simulink model "simu"  (R2019b)
settings: Solver=VariableStepAuto  StartTime=0.0  StopTime=1  RelTol=1e-3
(part 2 of 2)

== matlab function simu/Robot Torque  ==
  data: d1 input; te11 output; d2 input; d3 input; d4 input; L2 input; L3 input; L4 input; theta input; theta_dot input; theta_ddot input; mm input; II input; te22 output; te33 output; M output; G output; V output
function [te11,te22,te33,M,G,V] = fcn(d1,d2,d3,d4,L2,L3,L4,theta,theta_dot,theta_ddot,mm,II)
    theta1 = theta(1); theta2 = theta(2); theta3 = theta(3);
    theta1_dot = theta_dot(1); theta2_dot = theta_dot(2); theta3_dot = theta_dot(3);
    theta1_ddot = theta_ddot(1); theta2_ddot = theta_ddot(2); theta3_ddot = theta_ddot(3);
    m1 = mm(1); m2 =mm(2); m3 = mm(3); m4 = mm(4); m5 = mm(5);
    I1 = II(1); I2 = II(2); I3 = II(3); I4 = II(4); I5 = II(5);
    g = 9.8;
    te11 = 2*I1*theta1_ddot + 2*I2*theta1_ddot + 2*I3*theta1_ddot + 2*I4*theta1_ddot + 2*I5*theta1_ddot + (d2^2*m2*theta1_ddot)/2 + d2^2*m3*theta1_ddot + d2^2*m4*theta1_ddot + 2*d3^2*m3*theta1_ddot + d2^2*m5*theta1_ddot + d3^2*m4*theta1_ddot + d3^2*m5*theta1_ddot + 2*d4^2*m4*theta1_ddot + d4^2*m5*theta1_ddot + (5*L2^2*m3*theta1_ddot)/8 - (L2^2*m3*theta2_ddot)/4 + (L2^2*m4*theta1_ddot)/2 + (L2^2*m5*theta1_ddot)/2 + (5*L3^2*m4*theta1_ddot)/8 - (L3^2*m4*theta2_ddot)/4 + (L3^2*m5*theta1_ddot)/2 - (L3^2*m4*theta3_ddot)/4 + (5*L4^2*m5*theta1_ddot)/8 - (L4^2*m5*theta2_ddot)/4 - (L4^2*m5*theta3_ddot)/4 - (L2^2*m3*theta2_dot^2*sin(theta1 + theta2))/4 + (L3^2*m4*theta2_ddot*cos(theta1 + theta2 + theta3))/4 + (L3^2*m4*theta3_ddot*cos(theta1 + theta2 + theta3))/4 + (L4^2*m5*theta2_ddot*cos(theta1 + theta2 + theta3))/4 + (L4^2*m5*theta3_ddot*cos(theta1 + theta2 + theta3))/4 + (d2^2*m2*theta2_ddot*cos(theta1 - theta2))/2 - (d2^2*m2*theta2_dot^2*sin(theta1 + theta2))/2 - (d3^2*m3*theta1_dot^2*sin(theta1 + theta2))/2 + (L2^2*m3*theta1_ddot*cos(2*theta2))/2 + (L2^2*m4*theta1_ddot*cos(2*theta2))/2 + (L2^2*m5*theta1_ddot*cos(2*theta2))/2 + 2*d4^2*m4*theta1_ddot*cos(theta1 + theta2 + theta3) - (L2*g*m3*cos(theta1 + theta2))/2 - (L2*g*m4*cos(theta1 + theta2))/2 - (L2*g*m5*cos(theta1 + theta2))/2 + (d2^2*m2*theta1_ddot*cos(2*theta2))/2 - (d2*g*m2*sin(theta1 + theta2))/2 + (L2^2*m3*theta1_ddot*cos(2*theta2 + 2*theta3))/8 - (L2^2*m3*theta2_ddot*cos(2*theta2 + 2*theta3))/4 + (5*L3^2*m4*theta1_ddot*cos(2*theta2 + 2*theta3))/8 - (L3^2*m4*theta2_ddot*cos(2*theta2 + 2*theta3))/4 + (L3^2*m5*theta1_ddot*cos(2*theta2 + 2*theta3))/2 - (L3^2*m4*theta3_ddot*cos(2*theta2 + 2*theta3))/4 + (5*L4^2*m5*theta1_ddot*cos(2*theta2 + 2*theta3))/8 - (L4^2*m5*theta2_ddot*cos(2*theta2 + 2*theta3))/4 - (L4^2*m5*theta3_ddot*cos(2*theta2 + 2*theta3))/4 + (L2^2*m3*theta2_dot^2*sin(theta1 - theta2))/4 + (L3^2*m4*theta2_ddot*cos(theta2 - theta1 + theta3))/4 + (L3^2*m4*theta3_ddot*cos(theta2 - theta1 + theta3))/4 + (L4^2*m5*theta2_ddot*cos(theta2 - theta1 + theta3))/4 + (L4^2*m5*theta3_ddot*cos(theta2 - theta1 + theta3))/4 + (L2^2*m3*theta2_dot^2*sin(theta1 + theta2 + theta3))/4 + (d2^2*m2*theta2_dot^2*sin(theta1 - theta2))/2 - d2*g*m2*sin(theta1) - d2*g*m3*sin(theta1) - d2*g*m4*sin(theta1) - 2*d3*g*m3*sin(theta1) - d2*g*m5*sin(theta1) - d3*g*m4*sin(theta1) - d3*g*m5*sin(theta1) - 2*d4*g*m4*sin(theta1) - d4*g*m5*sin(theta1) + d3^2*m3*theta1_ddot*cos(theta1 + theta2 + 2*theta3) - (L2*g*m3*cos(theta1 - theta2))/2 - (L2*g*m4*cos(theta1 - theta2))/2 - (L2*g*m5*cos(theta1 - theta2))/2 - d4^2*m4*theta1_dot^2*sin(theta1 + theta2 + theta3) + (L2^2*m3*theta2_ddot*cos(theta1 + theta2))/4 + (L2^2*m3*theta3_ddot*cos(theta1 + theta2))/4 - (L2*g*m3*cos(theta1 + theta2 + theta3))/4 - (3*L3*g*m4*cos(theta1 + theta2 + theta3))/4 - (L3*g*m5*cos(theta1 + theta2 + theta3))/2 - (3*L4*g*m5*cos(theta1 + theta2 + theta3))/4 + (d2^2*m2*theta2_ddot*cos(theta1 + theta2))/2 + d3^2*m3*theta1_ddot*cos(theta1 + theta2) + (d2*g*m2*sin(theta1 - theta2))/2 + (L2^2*m3*theta2_dot^2*sin(2*theta2 + 2*theta3))/2 + (L3^2*m4*theta2_dot^2*sin(2*theta2 + 2*theta3))/2 + (L3^2*m4*theta3_dot^2*sin(2*theta2 + 2*theta3))/2 + (L4^2*m5*theta2_dot^2*sin(2*theta2 + 2*theta3))/2 + (L4^2*m5*theta3_dot^2*sin(2*theta2 + 2*theta3))/2 - (L2*L3*m4*theta2_ddot)/4 - (L2*L4*m5*theta2_ddot)/4 + L3*L4*m5*theta1_ddot - (L3*L4*m5*theta2_ddot)/4 - (L3*L4*m5*theta3_ddot)/4 + (L2^2*m3*theta2_dot^2*sin(theta2 - theta1 + theta3))/4 - (d3^2*m3*theta1_dot^2*sin(theta1 + theta2 + 2*theta3))/2 + (L2^2*m3*theta2_ddot*cos(theta1 - theta2))/4 + (L2^2*m3*theta3_ddot*cos(theta1 - theta2))/4 - (L2*g*m3*cos(theta2 - theta1 + theta3))/4 - (3*L3*g*m4*cos(theta2 - theta1 + theta3))/4 - (L3*g*m5*cos(theta2 - theta1 + theta3))/2 - (3*L4*g*m5*cos(theta2 - theta1 + theta3))/4 - d3^2*m3*theta1_dot*theta2_dot*sin(theta1 + theta2 + 2*theta3) - 2*d3^2*m3*theta1_dot*theta3_dot*sin(theta1 + theta2 + 2*theta3) + (L2*d2*m3*theta2_ddot*sin(theta1 - theta2))/4 + (L2*d2*m3*theta3_ddot*sin(theta1 - theta2))/4 - (L2*d2*m3*theta1_ddot*sin(2*theta2 + theta3))/2 + (L2*d3*m3*theta2_ddot*sin(theta1 - theta3))/4 + (L3*d2*m4*theta2_ddot*sin(theta1 - theta2))/4 - (L2*d3*m3*theta1_ddot*sin(theta2 + 2*theta3))/2 + (L2*d3*m3*theta3_ddot*sin(theta1 - theta3))/4 + (L3*d2*m4*theta3_ddot*sin(theta1 - theta2))/4 - (L3*d2*m4*theta1_ddot*sin(2*theta2 + theta3))/2 + (L3*d3*m4*theta2_ddot*sin(theta1 - theta3))/4 + (L4*d2*m5*theta2_ddot*sin(theta1 - theta2))/4 - (L3*d3*m4*theta1_ddot*sin(theta2 + 2*theta3))/2 + (L3*d3*m4*theta3_ddot*sin(theta1 - theta3))/4 + (L4*d2*m5*theta3_ddot*sin(theta1 - theta2))/4 - (L4*d2*m5*theta1_ddot*sin(2*theta2 + theta3))/2 + (L4*d3*m5*theta2_ddot*sin(theta1 - theta3))/4 - (L4*d3*m5*theta1_ddot*sin(theta2 + 2*theta3))/2 + (L4*d3*m5*theta3_ddot*sin(theta1 - theta3))/4 + 2*d2*d3*m3*theta1_ddot*cos(theta2 - theta3) + 2*d2*d3*m4*theta1_ddot*cos(theta2 - theta3) + 2*d2*d3*m5*theta1_ddot*cos(theta2 - theta3) - (L2^2*m3*theta2_dot*theta3_dot*sin(theta1 + theta2))/4 - (d2*d3*m3*theta1_dot^2*sin(theta1 + theta3))/2 - (d2*d4*m4*theta1_dot^2*sin(theta1 + theta3))/2 - (d3*d4*m4*theta1_dot^2*sin(theta1 + theta2))/2 - L2*d3*m3*theta2_dot^2*cos(theta2) - L2*d3*m4*theta2_dot^2*cos(theta2) - (L3*d4*m4*theta1_dot^2*cos(theta1))/2 - L2*d3*m5*theta2_dot^2*cos(theta2) - L3*d3*m4*theta2_dot^2*cos(theta2) - L3*d2*m4*theta3_dot^2*cos(theta3) - L3*d3*m5*theta2_dot^2*cos(theta2) - L3*d2*m5*theta3_dot^2*cos(theta3) - L4*d3*m5*theta2_dot^2*cos(theta2) - L4*d2*m5*theta3_dot^2*cos(theta3) - L2*d3*m3*theta2_dot^2*cos(theta1 + 2*theta2 + 2*theta3) - L2*d4*m4*theta2_dot^2*cos(theta1 + 2*theta2 + 2*theta3) - (L3*d4*m4*theta1_dot^2*cos(theta1 + 2*theta2 + 2*theta3))/2 - L3*d4*m4*theta2_dot^2*cos(theta1 + 2*theta2 + 2*theta3) - L3*d4*m4*theta3_dot^2*cos(theta1 + 2*theta2 + 2*theta3) - d3^2*m3*theta1_dot*theta2_dot*sin(theta1 + theta2) - (L2*L3*m4*theta2_ddot*cos(2*theta2 + 2*theta3))/4 - (L2*L4*m5*theta2_ddot*cos(2*theta2 + 2*theta3))/4 + L3*L4*m5*theta1_ddot*cos(2*theta2 + 2*theta3) - (L3*L4*m5*theta2_ddot*cos(2*theta2 + 2*theta3))/4 - (L3*L4*m5*theta3_ddot*cos(2*theta2 + 2*theta3))/4 + (L2*L3*m4*theta2_dot^2*sin(theta1 - theta2))/4 + (L2*L4*m5*theta2_dot^2*sin(theta1 - theta2))/4 + (L3*L4*m5*theta2_ddot*cos(theta2 - theta1 + theta3))/4 + (L3*L4*m5*theta3_ddot*cos(theta2 - theta1 + theta3))/4 - (L2*d2*m3*theta2_dot^2*cos(theta1 - theta2))/4 - (L3*d2*m4*theta2_dot^2*cos(theta1 - theta2))/4 - (L2*d3*m3*theta3_dot^2*cos(theta1 - theta3))/4 - (L4*d2*m5*theta2_dot^2*cos(theta1 - theta2))/4 - (L3*d3*m4*theta3_dot^2*cos(theta1 - theta3))/4 - (L4*d3*m5*theta3_dot^2*cos(theta1 - theta3))/4 + (L2*L3*m4*theta2_dot^2*sin(theta1 + theta2 + theta3))/4 + (L2*L4*m5*theta2_dot^2*sin(theta1 + theta2 + theta3))/4 + (L2^2*m3*theta2_dot*theta3_dot*sin(theta1 - theta2))/4 - L2*d3*m3*theta1_ddot*sin(theta1 + 2*theta2 + theta3) - L2*d4*m4*theta1_ddot*sin(theta1 + 2*theta2 + theta3) + (L2*L3*m4*theta2_ddot*cos(theta1 + theta2))/4 + (L2*L3*m4*theta3_ddot*cos(theta1 + theta2))/4 + (L2*L4*m5*theta2_ddot*cos(theta1 + theta2))/4 + (L2*L4*m5*theta3_ddot*cos(theta1 + theta2))/4 + d2*d3*m3*theta1_ddot*cos(theta1 + 2*theta2 + theta3) + d2*d4*m4*theta1_ddot*cos(theta1 + 2*theta2 + theta3) + d3*d4*m4*theta1_ddot*cos(theta1 + theta2 + 2*theta3) + (L2^2*m3*theta2_dot*theta3_dot*sin(theta1 + theta2 + theta3))/4 - L2^2*m3*theta1_dot*theta2_dot*sin(2*theta2) - L2^2*m4*theta1_dot*theta2_dot*sin(2*theta2) - L2^2*m5*theta1_dot*theta2_dot*sin(2*theta2) - 2*d4^2*m4*theta1_dot*theta2_dot*sin(theta1 + theta2 + theta3) - 2*d4^2*m4*theta1_dot*theta3_dot*sin(theta1 + theta2 + theta3) + (L2*d2*m3*theta2_ddot*sin(theta1 + theta2))/4 + (L2*d2*m3*theta3_ddot*sin(theta1 + theta2))/4 - L2*d3*m3*theta1_ddot*sin(theta1 + theta3) + (L2*d3*m3*theta2_ddot*sin(theta1 + theta3))/4 + (L3*d2*m4*theta2_ddot*sin(theta1 + theta2))/4 - (L2*d3*m3*theta2_ddot*sin(theta2 + theta3))/2 + (L2*d3*m3*theta3_ddot*sin(theta1 + theta3))/4 - L2*d4*m4*theta1_ddot*sin(theta1 + theta3) + (L3*d2*m4*theta3_ddot*sin(theta1 + theta2))/4 - (L2*d3*m3*theta3_ddot*sin(theta2 + theta3))/2 + (L3*d3*m4*theta2_ddot*sin(theta1 + theta3))/4 + (L4*d2*m5*theta2_ddot*sin(theta1 + theta2))/4 - L2*d4*m4*theta2_ddot*sin(theta2 + theta3) + (L3*d3*m4*theta3_ddot*sin(theta1 + theta3))/4 + (L4*d2*m5*theta3_ddot*sin(theta1 + theta2))/4 - L2*d4*m5*theta2_ddot*sin(theta2 + theta3) - (3*L3*d4*m4*theta2_ddot*sin(theta2 + theta3))/2 + (L4*d3*m5*theta2_ddot*sin(theta1 + theta3))/4 - (3*L3*d4*m4*theta3_ddot*sin(theta2 + theta3))/2 - L3*d4*m5*theta2_ddot*sin(theta2 + theta3) + (L4*d3*m5*theta3_ddot*sin(theta1 + theta3))/4 - L3*d4*m5*theta3_ddot*sin(theta2 + theta3) - L4*d4*m5*theta2_ddot*sin(theta2 + theta3) - L4*d4*m5*theta3_ddot*sin(theta2 + theta3) + L2*L3*m4*theta1_ddot*cos(theta3) + L2*L3*m5*theta1_ddot*cos(theta3) + L2*L4*m5*theta1_ddot*cos(theta3) + (L2*L3*m4*theta2_dot^2*sin(2*theta2 + 2*theta3))/2 + (L2*L4*m5*theta2_dot^2*sin(2*theta2 + 2*theta3))/2 + (L3*L4*m5*theta2_dot^2*sin(2*theta2 + 2*theta3))/2 + (L3*L4*m5*theta3_dot^2*sin(2*theta2 + 2*theta3))/2 + d2*d3*m3*theta1_ddot*cos(theta1 + theta3) + d2*d4*m4*theta1_ddot*cos(theta1 + theta3) + d3*d4*m4*theta1_ddot*cos(theta1 + theta2) - d2^2*m2*theta1_dot*theta2_dot*sin(2*theta2) + (L2*L3*m4*theta2_dot^2*sin(theta2 - theta1 + theta3))/4 + (L2*L4*m5*theta2_dot^2*sin(theta2 - theta1 + theta3))/4 - (L2*d3*m3*theta1_dot^2*cos(theta1 + 2*theta2 + theta3))/2 - (L2*d4*m4*theta1_dot^2*cos(theta1 + 2*theta2 + theta3))/2 + (L2*d2*m3*theta1_ddot*sin(theta3))/2 + (L2*d3*m3*theta1_ddot*sin(theta2))/2 + (L2*d3*m3*theta2_ddot*sin(theta1))/2 - L2*d2*m3*theta2_ddot*sin(theta3) - L2*d3*m3*theta2_ddot*sin(theta2) - L2*d2*m4*theta2_ddot*sin(theta3) - L2*d3*m4*theta2_ddot*sin(theta2) + (L2*d4*m4*theta2_ddot*sin(theta1))/2 + (L3*d2*m4*theta1_ddot*sin(theta3))/2 + (L3*d3*m4*theta1_ddot*sin(theta2))/2 - L3*d4*m4*theta1_ddot*sin(theta1) - L2*d2*m5*theta2_ddot*sin(theta3) - L2*d3*m5*theta2_ddot*sin(theta2) - L3*d2*m4*theta2_ddot*sin(theta3) - L3*d3*m4*theta2_ddot*sin(theta2) + L3*d4*m4*theta2_ddot*sin(theta1) - L3*d2*m4*theta3_ddot*sin(theta3) - L3*d2*m5*theta2_ddot*sin(theta3) - L3*d3*m4*theta3_ddot*sin(theta2) - L3*d3*m5*theta2_ddot*sin(theta2) + L3*d4*m4*theta3_ddot*sin(theta1) + (L4*d2*m5*theta1_ddot*sin(theta3))/2 + (L4*d3*m5*theta1_ddot*sin(theta2))/2 - L3*d2*m5*theta3_ddot*sin(theta3) - L3*d3*m5*theta3_ddot*sin(theta2) - L4*d2*m5*theta2_ddot*sin(theta3) - L4*d3*m5*theta2_ddot*sin(theta2) + (L4*d4*m5*theta2_ddot*sin(theta1))/2 - L4*d2*m5*theta3_ddot*sin(theta3) - L4*d3*m5*theta3_ddot*sin(theta2) + (L4*d4*m5*theta3_ddot*sin(theta1))/2 - (L2^2*m3*theta1_dot*theta2_dot*sin(2*theta2 + 2*theta3))/4 - (L2^2*m3*theta1_dot*theta3_dot*sin(2*theta2 + 2*theta3))/4 + (L2^2*m3*theta2_dot*theta3_dot*sin(2*theta2 + 2*theta3))/2 - (5*L3^2*m4*theta1_dot*theta2_dot*sin(2*theta2 + 2*theta3))/4 - (5*L3^2*m4*theta1_dot*theta3_dot*sin(2*theta2 + 2*theta3))/4 - L3^2*m5*theta1_dot*theta2_dot*sin(2*theta2 + 2*theta3) + L3^2*m4*theta2_dot*theta3_dot*sin(2*theta2 + 2*theta3) - L3^2*m5*theta1_dot*theta3_dot*sin(2*theta2 + 2*theta3) - (5*L4^2*m5*theta1_dot*theta2_dot*sin(2*theta2 + 2*theta3))/4 - (5*L4^2*m5*theta1_dot*theta3_dot*sin(2*theta2 + 2*theta3))/4 + L4^2*m5*theta2_dot*theta3_dot*sin(2*theta2 + 2*theta3) - (L2*d3*m3*theta2_ddot*sin(theta1 + 2*theta2 + 2*theta3))/2 - (L2*d4*m4*theta2_ddot*sin(theta1 + 2*theta2 + 2*theta3))/2 - L3*d4*m4*theta1_ddot*sin(theta1 + 2*theta2 + 2*theta3) - (L3*d4*m4*theta2_ddot*sin(theta1 + 2*theta2 + 2*theta3))/2 - (L3*d4*m4*theta3_ddot*sin(theta1 + 2*theta2 + 2*theta3))/2 + 2*d2*d4*m4*theta1_ddot*cos(theta2) + 2*d2*d4*m5*theta1_ddot*cos(theta2) + 2*d3*d4*m4*theta1_ddot*cos(theta3) + 2*d3*d4*m5*theta1_ddot*cos(theta3) + (L2*L3*m4*theta2_ddot*cos(theta1 - theta2))/4 + (L2*L3*m4*theta3_ddot*cos(theta1 - theta2))/4 + L2*L3*m4*theta1_ddot*cos(2*theta2 + theta3) + (L2*L4*m5*theta2_ddot*cos(theta1 - theta2))/4 + L2*L3*m5*theta1_ddot*cos(2*theta2 + theta3) + (L2*L4*m5*theta3_ddot*cos(theta1 - theta2))/4 + L2*L4*m5*theta1_ddot*cos(2*theta2 + theta3) + (L2^2*m3*theta2_dot*theta3_dot*sin(theta2 - theta1 + theta3))/4 - (L2*L3*m4*theta2_dot^2*sin(theta1 + theta2))/4 - (L2*L4*m5*theta2_dot^2*sin(theta1 + theta2))/4 - (d2*d3*m3*theta1_dot^2*sin(theta1 + 2*theta2 + theta3))/2 - (d2*d4*m4*theta1_dot^2*sin(theta1 + 2*theta2 + theta3))/2 - (d3*d4*m4*theta1_dot^2*sin(theta1 + theta2 + 2*theta3))/2 + (L3*L4*m5*theta2_ddot*cos(theta1 + theta2 + theta3))/4 + (L3*L4*m5*theta3_ddot*cos(theta1 + theta2 + theta3))/4 + (L2*d2*m3*theta2_dot^2*cos(theta1 + theta2))/4 - (L2*d3*m3*theta1_dot^2*cos(theta1 + theta3))/2 + (L3*d2*m4*theta2_dot^2*cos(theta1 + theta2))/4 - (L2*d3*m3*theta2_dot^2*cos(theta2 + theta3))/2 + (L2*d3*m3*theta3_dot^2*cos(theta1 + theta3))/4 - (L2*d4*m4*theta1_dot^2*cos(theta1 + theta3))/2 - (L2*d3*m3*theta3_dot^2*cos(theta2 + theta3))/2 + (L4*d2*m5*theta2_dot^2*cos(theta1 + theta2))/4 - L2*d4*m4*theta2_dot^2*cos(theta2 + theta3) + (L3*d3*m4*theta3_dot^2*cos(theta1 + theta3))/4 - L2*d4*m5*theta2_dot^2*cos(theta2 + theta3) - (3*L3*d4*m4*theta2_dot^2*cos(theta2 + theta3))/2 - (3*L3*d4*m4*theta3_dot^2*cos(theta2 + theta3))/2 - L3*d4*m5*theta2_dot^2*cos(theta2 + theta3) + (L4*d3*m5*theta3_dot^2*cos(theta1 + theta3))/4 - L3*d4*m5*theta3_dot^2*cos(theta2 + theta3) - L4*d4*m5*theta2_dot^2*cos(theta2 + theta3) - L4*d4*m5*theta3_dot^2*cos(theta2 + theta3) - (L2*L3*m4*theta2_dot*theta3_dot*sin(theta1 + theta2))/4 - (L2*L4*m5*theta2_dot*theta3_dot*sin(theta1 + theta2))/4 - 2*d2*d3*m3*theta1_dot*theta2_dot*sin(theta1 + 2*theta2 + theta3) - d2*d3*m3*theta1_dot*theta3_dot*sin(theta1 + 2*theta2 + theta3) - 2*d2*d4*m4*theta1_dot*theta2_dot*sin(theta1 + 2*theta2 + theta3) - d2*d4*m4*theta1_dot*theta3_dot*sin(theta1 + 2*theta2 + theta3) - d3*d4*m4*theta1_dot*theta2_dot*sin(theta1 + theta2 + 2*theta3) - 2*d3*d4*m4*theta1_dot*theta3_dot*sin(theta1 + theta2 + 2*theta3) + (L2*d2*m3*theta2_dot*theta3_dot*cos(theta1 + theta2))/4 - L2*d3*m3*theta1_dot*theta3_dot*cos(theta1 + theta3) + (L2*d3*m3*theta2_dot*theta3_dot*cos(theta1 + theta3))/4 + (L3*d2*m4*theta2_dot*theta3_dot*cos(theta1 + theta2))/4 - L2*d3*m3*theta2_dot*theta3_dot*cos(theta2 + theta3) - L2*d4*m4*theta1_dot*theta3_dot*cos(theta1 + theta3) + (L3*d3*m4*theta2_dot*theta3_dot*cos(theta1 + theta3))/4 + (L4*d2*m5*theta2_dot*theta3_dot*cos(theta1 + theta2))/4 - L2*d4*m4*theta2_dot*theta3_dot*cos(theta2 + theta3) - L2*d4*m5*theta2_dot*theta3_dot*cos(theta2 + theta3) - 3*L3*d4*m4*theta2_dot*theta3_dot*cos(theta2 + theta3) + (L4*d3*m5*theta2_dot*theta3_dot*cos(theta1 + theta3))/4 - 2*L3*d4*m5*theta2_dot*theta3_dot*cos(theta2 + theta3) - 2*L4*d4*m5*theta2_dot*theta3_dot*cos(theta2 + theta3) - L2*L3*m4*theta1_dot*theta3_dot*sin(theta3) - L2*L3*m5*theta1_dot*theta3_dot*sin(theta3) - L2*L4*m5*theta1_dot*theta3_dot*sin(theta3) - d2*d3*m3*theta1_dot*theta3_dot*sin(theta1 + theta3) - d3*d4*m4*theta1_dot*theta2_dot*sin(theta1 + theta2) - d2*d4*m4*theta1_dot*theta3_dot*sin(theta1 + theta3) + (L2*d3*m3*theta1_dot*theta2_dot*cos(theta2))/2 + (L2*d2*m3*theta1_dot*theta3_dot*cos(theta3))/2 - L2*d2*m3*theta2_dot*theta3_dot*cos(theta3) + (L3*d3*m4*theta1_dot*theta2_dot*cos(theta2))/2 - L2*d2*m4*theta2_dot*theta3_dot*cos(theta3) + (L3*d2*m4*theta1_dot*theta3_dot*cos(theta3))/2 - L2*d2*m5*theta2_dot*theta3_dot*cos(theta3) - L3*d2*m4*theta2_dot*theta3_dot*cos(theta3) - L3*d3*m4*theta2_dot*theta3_dot*cos(theta2) + (L4*d3*m5*theta1_dot*theta2_dot*cos(theta2))/2 - L3*d2*m5*theta2_dot*theta3_dot*cos(theta3) - L3*d3*m5*theta2_dot*theta3_dot*cos(theta2) + (L4*d2*m5*theta1_dot*theta3_dot*cos(theta3))/2 - L4*d2*m5*theta2_dot*theta3_dot*cos(theta3) - L4*d3*m5*theta2_dot*theta3_dot*cos(theta2) - L2*d3*m3*theta2_dot*theta3_dot*cos(theta1 + 2*theta2 + 2*theta3) - 2*L3*d4*m4*theta1_dot*theta2_dot*cos(theta1 + 2*theta2 + 2*theta3) - L2*d4*m4*theta2_dot*theta3_dot*cos(theta1 + 2*theta2 + 2*theta3) - 2*L3*d4*m4*theta1_dot*theta3_dot*cos(theta1 + 2*theta2 + 2*theta3) - 2*L3*d4*m4*theta2_dot*theta3_dot*cos(theta1 + 2*theta2 + 2*theta3) - 2*d2*d4*m4*theta1_dot*theta2_dot*sin(theta2) - 2*d2*d4*m5*theta1_dot*theta2_dot*sin(theta2) - 2*d3*d4*m4*theta1_dot*theta3_dot*sin(theta3) - 2*d3*d4*m5*theta1_dot*theta3_dot*sin(theta3) + (L2*L3*m4*theta2_dot*theta3_dot*sin(theta1 - theta2))/4 - 2*L2*L3*m4*theta1_dot*theta2_dot*sin(2*theta2 + theta3) - L2*L3*m4*theta1_dot*theta3_dot*sin(2*theta2 + theta3) - 2*L2*L3*m5*theta1_dot*theta2_dot*sin(2*theta2 + theta3) + (L2*L4*m5*theta2_dot*theta3_dot*sin(theta1 - theta2))/4 - L2*L3*m5*theta1_dot*theta3_dot*sin(2*theta2 + theta3) - 2*L2*L4*m5*theta1_dot*theta2_dot*sin(2*theta2 + theta3) - L2*L4*m5*theta1_dot*theta3_dot*sin(2*theta2 + theta3) - (L2*d2*m3*theta2_dot*theta3_dot*cos(theta1 - theta2))/4 - L2*d2*m3*theta1_dot*theta2_dot*cos(2*theta2 + theta3) - (L2*d2*m3*theta1_dot*theta3_dot*cos(2*theta2 + theta3))/2 - (L2*d3*m3*theta1_dot*theta2_dot*cos(theta2 + 2*theta3))/2 - (L2*d3*m3*theta2_dot*theta3_dot*cos(theta1 - theta3))/4 - (L3*d2*m4*theta2_dot*theta3_dot*cos(theta1 - theta2))/4 - L2*d3*m3*theta1_dot*theta3_dot*cos(theta2 + 2*theta3) - L3*d2*m4*theta1_dot*theta2_dot*cos(2*theta2 + theta3) - (L3*d2*m4*theta1_dot*theta3_dot*cos(2*theta2 + theta3))/2 - (L3*d3*m4*theta1_dot*theta2_dot*cos(theta2 + 2*theta3))/2 - (L3*d3*m4*theta2_dot*theta3_dot*cos(theta1 - theta3))/4 - (L4*d2*m5*theta2_dot*theta3_dot*cos(theta1 - theta2))/4 - L3*d3*m4*theta1_dot*theta3_dot*cos(theta2 + 2*theta3) - L4*d2*m5*theta1_dot*theta2_dot*cos(2*theta2 + theta3) - (L4*d2*m5*theta1_dot*theta3_dot*cos(2*theta2 + theta3))/2 - (L4*d3*m5*theta1_dot*theta2_dot*cos(theta2 + 2*theta3))/2 - (L4*d3*m5*theta2_dot*theta3_dot*cos(theta1 - theta3))/4 - L4*d3*m5*theta1_dot*theta3_dot*cos(theta2 + 2*theta3) + (L2*L3*m4*theta2_dot*theta3_dot*sin(theta1 + theta2 + theta3))/4 + (L2*L4*m5*theta2_dot*theta3_dot*sin(theta1 + theta2 + theta3))/4 - 2*d2*d3*m3*theta1_dot*theta2_dot*sin(theta2 - theta3) + 2*d2*d3*m3*theta1_dot*theta3_dot*sin(theta2 - theta3) - 2*d2*d3*m4*theta1_dot*theta2_dot*sin(theta2 - theta3) + 2*d2*d3*m4*theta1_dot*theta3_dot*sin(theta2 - theta3) - 2*d2*d3*m5*theta1_dot*theta2_dot*sin(theta2 - theta3) + 2*d2*d3*m5*theta1_dot*theta3_dot*sin(theta2 - theta3) + (L2*L3*m4*theta2_dot*theta3_dot*sin(2*theta2 + 2*theta3))/2 - 2*L3*L4*m5*theta1_dot*theta2_dot*sin(2*theta2 + 2*theta3) + (L2*L4*m5*theta2_dot*theta3_dot*sin(2*theta2 + 2*theta3))/2 - 2*L3*L4*m5*theta1_dot*theta3_dot*sin(2*theta2 + 2*theta3) + L3*L4*m5*theta2_dot*theta3_dot*sin(2*theta2 + 2*theta3) + (L2*L3*m4*theta2_dot*theta3_dot*sin(theta2 - theta1 + theta3))/4 + (L2*L4*m5*theta2_dot*theta3_dot*sin(theta2 - theta1 + theta3))/4 - 2*L2*d3*m3*theta1_dot*theta2_dot*cos(theta1 + 2*theta2 + theta3) - L2*d3*m3*theta1_dot*theta3_dot*cos(theta1 + 2*theta2 + theta3) - 2*L2*d4*m4*theta1_dot*theta2_dot*cos(theta1 + 2*theta2 + theta3) - L2*d4*m4*theta1_dot*theta3_dot*cos(theta1 + 2*theta2 + theta3);
    te22 = 2*I2*theta2_ddot + 2*I3*theta2_ddot + 2*I3*theta3_ddot + 2*I4*theta2_ddot + 2*I4*theta3_ddot + 2*I5*theta2_ddot + 2*I5*theta3_ddot + d2^2*m2*theta2_ddot - (L2^2*m3*theta1_ddot)/4 + (5*L2^2*m3*theta2_ddot)/4 + (L2^2*m3*theta3_ddot)/4 + L2^2*m4*theta2_ddot - (L3^2*m4*theta1_ddot)/4 + L2^2*m5*theta2_ddot + (5*L3^2*m4*theta2_ddot)/4 + (5*L3^2*m4*theta3_ddot)/4 + L3^2*m5*theta2_ddot - (L4^2*m5*theta1_ddot)/4 + L3^2*m5*theta3_ddot + (5*L4^2*m5*theta2_ddot)/4 + (5*L4^2*m5*theta3_ddot)/4 - (L2^2*m3*theta1_dot^2*sin(theta1 + theta2))/4 + (L2^2*m3*theta2_ddot*cos(theta1 + theta2 + theta3))/2 + (L2^2*m3*theta3_ddot*cos(theta1 + theta2 + theta3))/4 + (L3^2*m4*theta1_ddot*cos(theta1 + theta2 + theta3))/4 + (L3^2*m4*theta2_ddot*cos(theta1 + theta2 + theta3))/2 + (L3^2*m4*theta3_ddot*cos(theta1 + theta2 + theta3))/2 + (L4^2*m5*theta1_ddot*cos(theta1 + theta2 + theta3))/4 + (L4^2*m5*theta2_ddot*cos(theta1 + theta2 + theta3))/2 + (L4^2*m5*theta3_ddot*cos(theta1 + theta2 + theta3))/2 + (d2^2*m2*theta1_ddot*cos(theta1 - theta2))/2 - (d2^2*m2*theta1_dot^2*sin(theta1 + theta2))/2 + (d3^2*m3*theta1_dot^2*sin(theta1 + theta2))/2 - (L2*g*m3*cos(theta1 + theta2))/2 - (L2*g*m4*cos(theta1 + theta2))/2 - (L2*g*m5*cos(theta1 + theta2))/2 - (d2*g*m2*sin(theta1 + theta2))/2 - (L2^2*m3*theta1_ddot*cos(2*theta2 + 2*theta3))/4 - (L3^2*m4*theta1_ddot*cos(2*theta2 + 2*theta3))/4 - (L4^2*m5*theta1_ddot*cos(2*theta2 + 2*theta3))/4 - (L2^2*m3*theta1_dot^2*sin(theta1 - theta2))/4 - (L2^2*m3*theta2_ddot*cos(theta2 - theta1 + theta3))/2 - (L2^2*m3*theta3_ddot*cos(theta2 - theta1 + theta3))/4 + (L3^2*m4*theta1_ddot*cos(theta2 - theta1 + theta3))/4 - (L3^2*m4*theta2_ddot*cos(theta2 - theta1 + theta3))/2 - (L3^2*m4*theta3_ddot*cos(theta2 - theta1 + theta3))/2 + (L4^2*m5*theta1_ddot*cos(theta2 - theta1 + theta3))/4 - (L4^2*m5*theta2_ddot*cos(theta2 - theta1 + theta3))/2 - (L4^2*m5*theta3_ddot*cos(theta2 - theta1 + theta3))/2 - (L2^2*m3*theta2_dot^2*sin(theta1 + theta2 + theta3))/4 - (L2^2*m3*theta3_dot^2*sin(theta1 + theta2 + theta3))/4 - (L3^2*m4*theta1_dot^2*sin(theta1 + theta2 + theta3))/4 - (L3^2*m4*theta2_dot^2*sin(theta1 + theta2 + theta3))/4 - (L3^2*m4*theta3_dot^2*sin(theta1 + theta2 + theta3))/4 - (L4^2*m5*theta1_dot^2*sin(theta1 + theta2 + theta3))/4 - (L4^2*m5*theta2_dot^2*sin(theta1 + theta2 + theta3))/4 - (L4^2*m5*theta3_dot^2*sin(theta1 + theta2 + theta3))/4 - (d2^2*m2*theta1_dot^2*sin(theta1 - theta2))/2 + (L2*g*m3*cos(theta1 - theta2))/2 + (L2*g*m4*cos(theta1 - theta2))/2 + (L2*g*m5*cos(theta1 - theta2))/2 + (L2^2*m3*theta1_dot^2*sin(2*theta2))/2 + (L2^2*m4*theta1_dot^2*sin(2*theta2))/2 + (L2^2*m5*theta1_dot^2*sin(2*theta2))/2 + d4^2*m4*theta1_dot^2*sin(theta1 + theta2 + theta3) + (L2^2*m3*theta1_ddot*cos(theta1 + theta2))/4 - (L2*g*m3*cos(theta1 + theta2 + theta3))/4 - (3*L3*g*m4*cos(theta1 + theta2 + theta3))/4 - (L3*g*m5*cos(theta1 + theta2 + theta3))/2 - (3*L4*g*m5*cos(theta1 + theta2 + theta3))/4 + (d2^2*m2*theta1_dot^2*sin(2*theta2))/2 + (d2^2*m2*theta1_ddot*cos(theta1 + theta2))/2 - (d2*g*m2*sin(theta1 - theta2))/2 + (L2^2*m3*theta1_dot^2*sin(2*theta2 + 2*theta3))/8 + (5*L3^2*m4*theta1_dot^2*sin(2*theta2 + 2*theta3))/8 + (L3^2*m5*theta1_dot^2*sin(2*theta2 + 2*theta3))/2 + (5*L4^2*m5*theta1_dot^2*sin(2*theta2 + 2*theta3))/8 - (L2*L3*m4*theta1_ddot)/4 + 2*L2*L3*m4*theta2_ddot + L2*L3*m4*theta3_ddot + 2*L2*L3*m5*theta2_ddot - (L2*L4*m5*theta1_ddot)/4 + L2*L3*m5*theta3_ddot + 2*L2*L4*m5*theta2_ddot - (L3*L4*m5*theta1_ddot)/4 + L2*L4*m5*theta3_ddot + 2*L3*L4*m5*theta2_ddot + 2*L3*L4*m5*theta3_ddot + (L2^2*m3*theta2_dot^2*sin(theta2 - theta1 + theta3))/4 + (L2^2*m3*theta3_dot^2*sin(theta2 - theta1 + theta3))/4 + (L3^2*m4*theta1_dot^2*sin(theta2 - theta1 + theta3))/4 + (L3^2*m4*theta2_dot^2*sin(theta2 - theta1 + theta3))/4 + (L3^2*m4*theta3_dot^2*sin(theta2 - theta1 + theta3))/4 + (L4^2*m5*theta1_dot^2*sin(theta2 - theta1 + theta3))/4 + (L4^2*m5*theta2_dot^2*sin(theta2 - theta1 + theta3))/4 + (L4^2*m5*theta3_dot^2*sin(theta2 - theta1 + theta3))/4 + (d3^2*m3*theta1_dot^2*sin(theta1 + theta2 + 2*theta3))/2 + (L2^2*m3*theta1_ddot*cos(theta1 - theta2))/4 + (L2*g*m3*cos(theta2 - theta1 + theta3))/4 + (3*L3*g*m4*cos(theta2 - theta1 + theta3))/4 + (L3*g*m5*cos(theta2 - theta1 + theta3))/2 + (3*L4*g*m5*cos(theta2 - theta1 + theta3))/4 + (L2*d2*m3*theta1_ddot*sin(theta1 - theta2))/4 + (L2*d3*m3*theta1_ddot*sin(theta1 - theta3))/4 + (L3*d2*m4*theta1_ddot*sin(theta1 - theta2))/4 + (L3*d3*m4*theta1_ddot*sin(theta1 - theta3))/4 + (L4*d2*m5*theta1_ddot*sin(theta1 - theta2))/4 + (L4*d3*m5*theta1_ddot*sin(theta1 - theta3))/4 + (L2^2*m3*theta1_dot*theta3_dot*sin(theta1 + theta2))/4 + (d3*d4*m4*theta1_dot^2*sin(theta1 + theta2))/2 + (L2*d3*m3*theta1_dot^2*cos(theta1))/2 - (L2*d3*m3*theta1_dot^2*cos(theta2))/4 + (L2*d4*m4*theta1_dot^2*cos(theta1))/2 - (L3*d3*m4*theta1_dot^2*cos(theta2))/4 + L3*d4*m4*theta1_dot^2*cos(theta1) - (L4*d3*m5*theta1_dot^2*cos(theta2))/4 + (L4*d4*m5*theta1_dot^2*cos(theta1))/2 - (L2*d3*m3*theta1_dot^2*cos(theta1 + 2*theta2 + 2*theta3))/2 - (L2*d4*m4*theta1_dot^2*cos(theta1 + 2*theta2 + 2*theta3))/2 + (L3*d4*m4*theta1_dot^2*cos(theta1 + 2*theta2 + 2*theta3))/2 - (L2*L3*m4*theta1_ddot*cos(2*theta2 + 2*theta3))/4 - (L2*L4*m5*theta1_ddot*cos(2*theta2 + 2*theta3))/4 - (L3*L4*m5*theta1_ddot*cos(2*theta2 + 2*theta3))/4 + d2*d4*m4*theta1_dot^2*sin(theta2) + d2*d4*m5*theta1_dot^2*sin(theta2) - (L2*L3*m4*theta1_dot^2*sin(theta1 - theta2))/4 - (L2*L4*m5*theta1_dot^2*sin(theta1 - theta2))/4 + L2*L3*m4*theta1_dot^2*sin(2*theta2 + theta3) + L2*L3*m5*theta1_dot^2*sin(2*theta2 + theta3) + L2*L4*m5*theta1_dot^2*sin(2*theta2 + theta3) - (L2*L3*m4*theta2_ddot*cos(theta2 - theta1 + theta3))/2 - (L2*L3*m4*theta3_ddot*cos(theta2 - theta1 + theta3))/4 - (L2*L4*m5*theta2_ddot*cos(theta2 - theta1 + theta3))/2 + (L3*L4*m5*theta1_ddot*cos(theta2 - theta1 + theta3))/4 - (L2*L4*m5*theta3_ddot*cos(theta2 - theta1 + theta3))/4 - (L3*L4*m5*theta2_ddot*cos(theta2 - theta1 + theta3))/2 - (L3*L4*m5*theta3_ddot*cos(theta2 - theta1 + theta3))/2 + (L2*d2*m3*theta1_dot^2*cos(theta1 - theta2))/4 + (L2*d3*m3*theta1_dot^2*cos(theta1 - theta3))/4 + (L3*d2*m4*theta1_dot^2*cos(theta1 - theta2))/4 + (L2*d2*m3*theta1_dot^2*cos(2*theta2 + theta3))/2 + (L2*d3*m3*theta1_dot^2*cos(theta2 + 2*theta3))/4 + (L3*d3*m4*theta1_dot^2*cos(theta1 - theta3))/4 + (L4*d2*m5*theta1_dot^2*cos(theta1 - theta2))/4 + (L3*d2*m4*theta1_dot^2*cos(2*theta2 + theta3))/2 + (L3*d3*m4*theta1_dot^2*cos(theta2 + 2*theta3))/4 + (L4*d3*m5*theta1_dot^2*cos(theta1 - theta3))/4 + (L4*d2*m5*theta1_dot^2*cos(2*theta2 + theta3))/2 + (L4*d3*m5*theta1_dot^2*cos(theta2 + 2*theta3))/4 - (L2*L3*m4*theta2_dot^2*sin(theta1 + theta2 + theta3))/4 - (L2*L3*m4*theta3_dot^2*sin(theta1 + theta2 + theta3))/4 - (L2*L4*m5*theta2_dot^2*sin(theta1 + theta2 + theta3))/4 - (L3*L4*m5*theta1_dot^2*sin(theta1 + theta2 + theta3))/4 - (L2*L4*m5*theta3_dot^2*sin(theta1 + theta2 + theta3))/4 - (L3*L4*m5*theta2_dot^2*sin(theta1 + theta2 + theta3))/4 - (L3*L4*m5*theta3_dot^2*sin(theta1 + theta2 + theta3))/4 - (L2^2*m3*theta1_dot*theta3_dot*sin(theta1 - theta2))/4 + d2*d3*m3*theta1_dot^2*sin(theta2 - theta3) + d2*d3*m4*theta1_dot^2*sin(theta2 - theta3) + d2*d3*m5*theta1_dot^2*sin(theta2 - theta3) + (L2*L3*m4*theta1_ddot*cos(theta1 + theta2))/4 + (L2*L4*m5*theta1_ddot*cos(theta1 + theta2))/4 - (L2^2*m3*theta1_dot*theta2_dot*sin(theta1 + theta2 + theta3))/2 - (L2^2*m3*theta1_dot*theta3_dot*sin(theta1 + theta2 + theta3))/4 - (L2^2*m3*theta2_dot*theta3_dot*sin(theta1 + theta2 + theta3))/2 - (L3^2*m4*theta1_dot*theta2_dot*sin(theta1 + theta2 + theta3))/2 - (L3^2*m4*theta1_dot*theta3_dot*sin(theta1 + theta2 + theta3))/2 - (L3^2*m4*theta2_dot*theta3_dot*sin(theta1 + theta2 + theta3))/2 - (L4^2*m5*theta1_dot*theta2_dot*sin(theta1 + theta2 + theta3))/2 - (L4^2*m5*theta1_dot*theta3_dot*sin(theta1 + theta2 + theta3))/2 - (L4^2*m5*theta2_dot*theta3_dot*sin(theta1 + theta2 + theta3))/2 + (L2*d2*m3*theta1_ddot*sin(theta1 + theta2))/4 + (L2*d3*m3*theta1_ddot*sin(theta1 + theta3))/4 + (L3*d2*m4*theta1_ddot*sin(theta1 + theta2))/4 - (L2*d3*m3*theta1_ddot*sin(theta2 + theta3))/2 + (L3*d3*m4*theta1_ddot*sin(theta1 + theta3))/4 + (L4*d2*m5*theta1_ddot*sin(theta1 + theta2))/4 - L2*d4*m4*theta1_ddot*sin(theta2 + theta3) - L2*d4*m5*theta1_ddot*sin(theta2 + theta3) - (3*L3*d4*m4*theta1_ddot*sin(theta2 + theta3))/2 + (L4*d3*m5*theta1_ddot*sin(theta1 + theta3))/4 - L3*d4*m5*theta1_ddot*sin(theta2 + theta3) - L4*d4*m5*theta1_ddot*sin(theta2 + theta3) + L3*L4*m5*theta1_dot^2*sin(2*theta2 + 2*theta3) + (L2*L3*m4*theta2_dot^2*sin(theta2 - theta1 + theta3))/4 + (L2*L3*m4*theta3_dot^2*sin(theta2 - theta1 + theta3))/4 + (L2*L4*m5*theta2_dot^2*sin(theta2 - theta1 + theta3))/4 + (L3*L4*m5*theta1_dot^2*sin(theta2 - theta1 + theta3))/4 + (L2*L4*m5*theta3_dot^2*sin(theta2 - theta1 + theta3))/4 + (L3*L4*m5*theta2_dot^2*sin(theta2 - theta1 + theta3))/4 + (L3*L4*m5*theta3_dot^2*sin(theta2 - theta1 + theta3))/4 + L2*d3*m3*theta1_dot^2*cos(theta1 + 2*theta2 + theta3) + L2*d4*m4*theta1_dot^2*cos(theta1 + 2*theta2 + theta3) + (L2*d3*m3*theta1_ddot*sin(theta1))/2 - L2*d2*m3*theta1_ddot*sin(theta3) - L2*d3*m3*theta1_ddot*sin(theta2) - L2*d2*m4*theta1_ddot*sin(theta3) - L2*d3*m4*theta1_ddot*sin(theta2) + (L2*d4*m4*theta1_ddot*sin(theta1))/2 - L2*d2*m5*theta1_ddot*sin(theta3) - L2*d3*m5*theta1_ddot*sin(theta2) - L3*d2*m4*theta1_ddot*sin(theta3) - L3*d3*m4*theta1_ddot*sin(theta2) + L3*d4*m4*theta1_ddot*sin(theta1) - L3*d2*m5*theta1_ddot*sin(theta3) - L3*d3*m5*theta1_ddot*sin(theta2) - L4*d2*m5*theta1_ddot*sin(theta3) - L4*d3*m5*theta1_ddot*sin(theta2) + (L4*d4*m5*theta1_ddot*sin(theta1))/2 + (L2^2*m3*theta1_dot*theta3_dot*sin(2*theta2 + 2*theta3))/2 - (L2*d3*m3*theta1_ddot*sin(theta1 + 2*theta2 + 2*theta3))/2 - (L2*d4*m4*theta1_ddot*sin(theta1 + 2*theta2 + 2*theta3))/2 - (L3*d4*m4*theta1_ddot*sin(theta1 + 2*theta2 + 2*theta3))/2 + (L2*L3*m4*theta1_ddot*cos(theta1 - theta2))/4 + (L2*L4*m5*theta1_ddot*cos(theta1 - theta2))/4 - (L2^2*m3*theta1_dot*theta2_dot*sin(theta2 - theta1 + theta3))/2 - (L2^2*m3*theta1_dot*theta3_dot*sin(theta2 - theta1 + theta3))/4 + (L2^2*m3*theta2_dot*theta3_dot*sin(theta2 - theta1 + theta3))/2 - (L3^2*m4*theta1_dot*theta2_dot*sin(theta2 - theta1 + theta3))/2 - (L3^2*m4*theta1_dot*theta3_dot*sin(theta2 - theta1 + theta3))/2 + (L3^2*m4*theta2_dot*theta3_dot*sin(theta2 - theta1 + theta3))/2 - (L4^2*m5*theta1_dot*theta2_dot*sin(theta2 - theta1 + theta3))/2 - (L4^2*m5*theta1_dot*theta3_dot*sin(theta2 - theta1 + theta3))/2 + (L4^2*m5*theta2_dot*theta3_dot*sin(theta2 - theta1 + theta3))/2 - (L2*L3*m4*theta1_dot^2*sin(theta1 + theta2))/4 - (L2*L4*m5*theta1_dot^2*sin(theta1 + theta2))/4 + d2*d3*m3*theta1_dot^2*sin(theta1 + 2*theta2 + theta3) + d2*d4*m4*theta1_dot^2*sin(theta1 + 2*theta2 + theta3) + (d3*d4*m4*theta1_dot^2*sin(theta1 + theta2 + 2*theta3))/2 + (L2*L3*m4*theta2_ddot*cos(theta1 + theta2 + theta3))/2 + (L2*L3*m4*theta3_ddot*cos(theta1 + theta2 + theta3))/4 + (L2*L4*m5*theta2_ddot*cos(theta1 + theta2 + theta3))/2 + (L3*L4*m5*theta1_ddot*cos(theta1 + theta2 + theta3))/4 + (L2*L4*m5*theta3_ddot*cos(theta1 + theta2 + theta3))/4 + (L3*L4*m5*theta2_ddot*cos(theta1 + theta2 + theta3))/2 + (L3*L4*m5*theta3_ddot*cos(theta1 + theta2 + theta3))/2 + (L2*d2*m3*theta1_dot^2*cos(theta1 + theta2))/4 + (L2*d3*m3*theta1_dot^2*cos(theta1 + theta3))/4 + (L3*d2*m4*theta1_dot^2*cos(theta1 + theta2))/4 + (L3*d3*m4*theta1_dot^2*cos(theta1 + theta3))/4 + (L4*d2*m5*theta1_dot^2*cos(theta1 + theta2))/4 + (L4*d3*m5*theta1_dot^2*cos(theta1 + theta3))/4 + (L2*L3*m4*theta1_dot*theta3_dot*sin(theta1 + theta2))/4 + (L2*L4*m5*theta1_dot*theta3_dot*sin(theta1 + theta2))/4 - (L2*d2*m3*theta1_dot*theta3_dot*cos(theta1 + theta2))/4 + (L2*d3*m3*theta1_dot*theta3_dot*cos(theta1 + theta3))/4 - (L3*d2*m4*theta1_dot*theta3_dot*cos(theta1 + theta2))/4 + (L3*d3*m4*theta1_dot*theta3_dot*cos(theta1 + theta3))/4 - (L4*d2*m5*theta1_dot*theta3_dot*cos(theta1 + theta2))/4 - L2*d4*m4*theta1_dot*theta3_dot*cos(theta2 + theta3) - L2*d4*m5*theta1_dot*theta3_dot*cos(theta2 + theta3) + (L4*d3*m5*theta1_dot*theta3_dot*cos(theta1 + theta3))/4 - L2*d2*m3*theta1_dot*theta3_dot*cos(theta3) - L2*d2*m4*theta1_dot*theta3_dot*cos(theta3) - L2*d2*m5*theta1_dot*theta3_dot*cos(theta3) - L3*d2*m4*theta1_dot*theta3_dot*cos(theta3) + L3*d3*m4*theta1_dot*theta3_dot*cos(theta2) - L3*d2*m5*theta1_dot*theta3_dot*cos(theta3) + L3*d3*m5*theta1_dot*theta3_dot*cos(theta2) - L4*d2*m5*theta1_dot*theta3_dot*cos(theta3) + L4*d3*m5*theta1_dot*theta3_dot*cos(theta2) - L2*d3*m3*theta1_dot*theta3_dot*cos(theta1 + 2*theta2 + 2*theta3) - L2*d4*m4*theta1_dot*theta3_dot*cos(theta1 + 2*theta2 + 2*theta3) - (L2*L3*m4*theta1_dot*theta3_dot*sin(theta1 - theta2))/4 - (L2*L4*m5*theta1_dot*theta3_dot*sin(theta1 - theta2))/4 + (L2*d2*m3*theta1_dot*theta3_dot*cos(theta1 - theta2))/4 - (L2*d3*m3*theta1_dot*theta3_dot*cos(theta1 - theta3))/4 + (L3*d2*m4*theta1_dot*theta3_dot*cos(theta1 - theta2))/4 - (L3*d3*m4*theta1_dot*theta3_dot*cos(theta1 - theta3))/4 + (L4*d2*m5*theta1_dot*theta3_dot*cos(theta1 - theta2))/4 - (L4*d3*m5*theta1_dot*theta3_dot*cos(theta1 - theta3))/4 - (L2*L3*m4*theta1_dot*theta2_dot*sin(theta1 + theta2 + theta3))/2 - (L2*L3*m4*theta1_dot*theta3_dot*sin(theta1 + theta2 + theta3))/4 - (L2*L3*m4*theta2_dot*theta3_dot*sin(theta1 + theta2 + theta3))/2 - (L2*L4*m5*theta1_dot*theta2_dot*sin(theta1 + theta2 + theta3))/2 - (L2*L4*m5*theta1_dot*theta3_dot*sin(theta1 + theta2 + theta3))/4 - (L3*L4*m5*theta1_dot*theta2_dot*sin(theta1 + theta2 + theta3))/2 - (L2*L4*m5*theta2_dot*theta3_dot*sin(theta1 + theta2 + theta3))/2 - (L3*L4*m5*theta1_dot*theta3_dot*sin(theta1 + theta2 + theta3))/2 - (L3*L4*m5*theta2_dot*theta3_dot*sin(theta1 + theta2 + theta3))/2 + (L2*L3*m4*theta1_dot*theta3_dot*sin(2*theta2 + 2*theta3))/2 + (L2*L4*m5*theta1_dot*theta3_dot*sin(2*theta2 + 2*theta3))/2 - (L2*L3*m4*theta1_dot*theta2_dot*sin(theta2 - theta1 + theta3))/2 - (L2*L3*m4*theta1_dot*theta3_dot*sin(theta2 - theta1 + theta3))/4 + (L2*L3*m4*theta2_dot*theta3_dot*sin(theta2 - theta1 + theta3))/2 - (L2*L4*m5*theta1_dot*theta2_dot*sin(theta2 - theta1 + theta3))/2 - (L2*L4*m5*theta1_dot*theta3_dot*sin(theta2 - theta1 + theta3))/4 - (L3*L4*m5*theta1_dot*theta2_dot*sin(theta2 - theta1 + theta3))/2 + (L2*L4*m5*theta2_dot*theta3_dot*sin(theta2 - theta1 + theta3))/2 - (L3*L4*m5*theta1_dot*theta3_dot*sin(theta2 - theta1 + theta3))/2 + (L3*L4*m5*theta2_dot*theta3_dot*sin(theta2 - theta1 + theta3))/2;
    te33 = 2*I3*theta2_ddot + 2*I3*theta3_ddot + 2*I4*theta2_ddot + 2*I4*theta3_ddot + 2*I5*theta2_ddot + 2*I5*theta3_ddot + (L2^2*m3*theta2_ddot)/4 + (L2^2*m3*theta3_ddot)/4 - (L3^2*m4*theta1_ddot)/4 + (5*L3^2*m4*theta2_ddot)/4 + (5*L3^2*m4*theta3_ddot)/4 + L3^2*m5*theta2_ddot - (L4^2*m5*theta1_ddot)/4 + L3^2*m5*theta3_ddot + (5*L4^2*m5*theta2_ddot)/4 + (5*L4^2*m5*theta3_ddot)/4 - (L2^2*m3*theta1_dot^2*sin(theta1 + theta2))/4 + (L2^2*m3*theta2_ddot*cos(theta1 + theta2 + theta3))/4 + (L3^2*m4*theta1_ddot*cos(theta1 + theta2 + theta3))/4 + (L3^2*m4*theta2_ddot*cos(theta1 + theta2 + theta3))/2 + (L3^2*m4*theta3_ddot*cos(theta1 + theta2 + theta3))/2 + (L4^2*m5*theta1_ddot*cos(theta1 + theta2 + theta3))/4 + (L4^2*m5*theta2_ddot*cos(theta1 + theta2 + theta3))/2 + (L4^2*m5*theta3_ddot*cos(theta1 + theta2 + theta3))/2 - (L3^2*m4*theta1_ddot*cos(2*theta2 + 2*theta3))/4 - (L4^2*m5*theta1_ddot*cos(2*theta2 + 2*theta3))/4 - (L2^2*m3*theta1_dot^2*sin(theta1 - theta2))/4 - (L2^2*m3*theta2_ddot*cos(theta2 - theta1 + theta3))/4 + (L3^2*m4*theta1_ddot*cos(theta2 - theta1 + theta3))/4 - (L3^2*m4*theta2_ddot*cos(theta2 - theta1 + theta3))/2 - (L3^2*m4*theta3_ddot*cos(theta2 - theta1 + theta3))/2 + (L4^2*m5*theta1_ddot*cos(theta2 - theta1 + theta3))/4 - (L4^2*m5*theta2_ddot*cos(theta2 - theta1 + theta3))/2 - (L4^2*m5*theta3_ddot*cos(theta2 - theta1 + theta3))/2 - (L3^2*m4*theta1_dot^2*sin(theta1 + theta2 + theta3))/4 - (L3^2*m4*theta2_dot^2*sin(theta1 + theta2 + theta3))/4 - (L3^2*m4*theta3_dot^2*sin(theta1 + theta2 + theta3))/4 - (L4^2*m5*theta1_dot^2*sin(theta1 + theta2 + theta3))/4 - (L4^2*m5*theta2_dot^2*sin(theta1 + theta2 + theta3))/4 - (L4^2*m5*theta3_dot^2*sin(theta1 + theta2 + theta3))/4 + d4^2*m4*theta1_dot^2*sin(theta1 + theta2 + theta3) + (L2^2*m3*theta1_ddot*cos(theta1 + theta2))/4 - (L2*g*m3*cos(theta1 + theta2 + theta3))/4 - (3*L3*g*m4*cos(theta1 + theta2 + theta3))/4 - (L3*g*m5*cos(theta1 + theta2 + theta3))/2 - (3*L4*g*m5*cos(theta1 + theta2 + theta3))/4 + (L2^2*m3*theta1_dot^2*sin(2*theta2 + 2*theta3))/8 + (5*L3^2*m4*theta1_dot^2*sin(2*theta2 + 2*theta3))/8 + (L3^2*m5*theta1_dot^2*sin(2*theta2 + 2*theta3))/2 + (5*L4^2*m5*theta1_dot^2*sin(2*theta2 + 2*theta3))/8 + L2*L3*m4*theta2_ddot + L2*L3*m5*theta2_ddot + L2*L4*m5*theta2_ddot - (L3*L4*m5*theta1_ddot)/4 + 2*L3*L4*m5*theta2_ddot + 2*L3*L4*m5*theta3_ddot + (L3^2*m4*theta1_dot^2*sin(theta2 - theta1 + theta3))/4 + (L3^2*m4*theta2_dot^2*sin(theta2 - theta1 + theta3))/4 + (L3^2*m4*theta3_dot^2*sin(theta2 - theta1 + theta3))/4 + (L4^2*m5*theta1_dot^2*sin(theta2 - theta1 + theta3))/4 + (L4^2*m5*theta2_dot^2*sin(theta2 - theta1 + theta3))/4 + (L4^2*m5*theta3_dot^2*sin(theta2 - theta1 + theta3))/4 + d3^2*m3*theta1_dot^2*sin(theta1 + theta2 + 2*theta3) + (L2^2*m3*theta1_ddot*cos(theta1 - theta2))/4 + (L2*g*m3*cos(theta2 - theta1 + theta3))/4 + (3*L3*g*m4*cos(theta2 - theta1 + theta3))/4 + (L3*g*m5*cos(theta2 - theta1 + theta3))/2 + (3*L4*g*m5*cos(theta2 - theta1 + theta3))/4 + (L2*d2*m3*theta1_ddot*sin(theta1 - theta2))/4 + (L2*d3*m3*theta1_ddot*sin(theta1 - theta3))/4 + (L3*d2*m4*theta1_ddot*sin(theta1 - theta2))/4 + (L3*d3*m4*theta1_ddot*sin(theta1 - theta3))/4 + (L4*d2*m5*theta1_ddot*sin(theta1 - theta2))/4 + (L4*d3*m5*theta1_ddot*sin(theta1 - theta3))/4 - (L2^2*m3*theta1_dot*theta2_dot*sin(theta1 + theta2))/4 + (L2*L3*m4*theta1_dot^2*sin(theta3))/2 + (L2*L3*m5*theta1_dot^2*sin(theta3))/2 + (L2*L4*m5*theta1_dot^2*sin(theta3))/2 + (d2*d3*m3*theta1_dot^2*sin(theta1 + theta3))/2 + (d2*d4*m4*theta1_dot^2*sin(theta1 + theta3))/2 - (L2*d2*m3*theta1_dot^2*cos(theta3))/4 - (L3*d2*m4*theta1_dot^2*cos(theta3))/4 + L3*d4*m4*theta1_dot^2*cos(theta1) - (L4*d2*m5*theta1_dot^2*cos(theta3))/4 + (L4*d4*m5*theta1_dot^2*cos(theta1))/2 + (L3*d4*m4*theta1_dot^2*cos(theta1 + 2*theta2 + 2*theta3))/2 - (L3*L4*m5*theta1_ddot*cos(2*theta2 + 2*theta3))/4 + d3*d4*m4*theta1_dot^2*sin(theta3) + d3*d4*m5*theta1_dot^2*sin(theta3) - (L2*L3*m4*theta1_dot^2*sin(theta1 - theta2))/4 - (L2*L4*m5*theta1_dot^2*sin(theta1 - theta2))/4 + (L2*L3*m4*theta1_dot^2*sin(2*theta2 + theta3))/2 + (L2*L3*m5*theta1_dot^2*sin(2*theta2 + theta3))/2 + (L2*L4*m5*theta1_dot^2*sin(2*theta2 + theta3))/2 - (L2*L3*m4*theta2_ddot*cos(theta2 - theta1 + theta3))/4 - (L2*L4*m5*theta2_ddot*cos(theta2 - theta1 + theta3))/4 + (L3*L4*m5*theta1_ddot*cos(theta2 - theta1 + theta3))/4 - (L3*L4*m5*theta2_ddot*cos(theta2 - theta1 + theta3))/2 - (L3*L4*m5*theta3_ddot*cos(theta2 - theta1 + theta3))/2 + (L2*d2*m3*theta1_dot^2*cos(theta1 - theta2))/4 + (L2*d3*m3*theta1_dot^2*cos(theta1 - theta3))/4 + (L3*d2*m4*theta1_dot^2*cos(theta1 - theta2))/4 + (L2*d2*m3*theta1_dot^2*cos(2*theta2 + theta3))/4 + (L2*d3*m3*theta1_dot^2*cos(theta2 + 2*theta3))/2 + (L3*d3*m4*theta1_dot^2*cos(theta1 - theta3))/4 + (L4*d2*m5*theta1_dot^2*cos(theta1 - theta2))/4 + (L3*d2*m4*theta1_dot^2*cos(2*theta2 + theta3))/4 + (L3*d3*m4*theta1_dot^2*cos(theta2 + 2*theta3))/2 + (L4*d3*m5*theta1_dot^2*cos(theta1 - theta3))/4 + (L4*d2*m5*theta1_dot^2*cos(2*theta2 + theta3))/4 + (L4*d3*m5*theta1_dot^2*cos(theta2 + 2*theta3))/2 - (L3*L4*m5*theta1_dot^2*sin(theta1 + theta2 + theta3))/4 - (L3*L4*m5*theta2_dot^2*sin(theta1 + theta2 + theta3))/4 - (L3*L4*m5*theta3_dot^2*sin(theta1 + theta2 + theta3))/4 + (L2^2*m3*theta1_dot*theta2_dot*sin(theta1 - theta2))/4 - d2*d3*m3*theta1_dot^2*sin(theta2 - theta3) - d2*d3*m4*theta1_dot^2*sin(theta2 - theta3) - d2*d3*m5*theta1_dot^2*sin(theta2 - theta3) + (L2*L3*m4*theta1_ddot*cos(theta1 + theta2))/4 + (L2*L4*m5*theta1_ddot*cos(theta1 + theta2))/4 - (L2^2*m3*theta1_dot*theta2_dot*sin(theta1 + theta2 + theta3))/4 - (L3^2*m4*theta1_dot*theta2_dot*sin(theta1 + theta2 + theta3))/2 - (L3^2*m4*theta1_dot*theta3_dot*sin(theta1 + theta2 + theta3))/2 - (L3^2*m4*theta2_dot*theta3_dot*sin(theta1 + theta2 + theta3))/2 - (L4^2*m5*theta1_dot*theta2_dot*sin(theta1 + theta2 + theta3))/2 - (L4^2*m5*theta1_dot*theta3_dot*sin(theta1 + theta2 + theta3))/2 - (L4^2*m5*theta2_dot*theta3_dot*sin(theta1 + theta2 + theta3))/2 + (L2*d2*m3*theta1_ddot*sin(theta1 + theta2))/4 + (L2*d3*m3*theta1_ddot*sin(theta1 + theta3))/4 + (L3*d2*m4*theta1_ddot*sin(theta1 + theta2))/4 - (L2*d3*m3*theta1_ddot*sin(theta2 + theta3))/2 + (L3*d3*m4*theta1_ddot*sin(theta1 + theta3))/4 + (L4*d2*m5*theta1_ddot*sin(theta1 + theta2))/4 - (3*L3*d4*m4*theta1_ddot*sin(theta2 + theta3))/2 + (L4*d3*m5*theta1_ddot*sin(theta1 + theta3))/4 - L3*d4*m5*theta1_ddot*sin(theta2 + theta3) - L4*d4*m5*theta1_ddot*sin(theta2 + theta3) + L3*L4*m5*theta1_dot^2*sin(2*theta2 + 2*theta3) + (L3*L4*m5*theta1_dot^2*sin(theta2 - theta1 + theta3))/4 + (L3*L4*m5*theta2_dot^2*sin(theta2 - theta1 + theta3))/4 + (L3*L4*m5*theta3_dot^2*sin(theta2 - theta1 + theta3))/4 + (L2*d3*m3*theta1_dot^2*cos(theta1 + 2*theta2 + theta3))/2 + (L2*d4*m4*theta1_dot^2*cos(theta1 + 2*theta2 + theta3))/2 - L3*d2*m4*theta1_ddot*sin(theta3) - L3*d3*m4*theta1_ddot*sin(theta2) + L3*d4*m4*theta1_ddot*sin(theta1) - L3*d2*m5*theta1_ddot*sin(theta3) - L3*d3*m5*theta1_ddot*sin(theta2) - L4*d2*m5*theta1_ddot*sin(theta3) - L4*d3*m5*theta1_ddot*sin(theta2) + (L4*d4*m5*theta1_ddot*sin(theta1))/2 - (L2^2*m3*theta1_dot*theta2_dot*sin(2*theta2 + 2*theta3))/2 - (L3*d4*m4*theta1_ddot*sin(theta1 + 2*theta2 + 2*theta3))/2 + (L2*L3*m4*theta1_ddot*cos(theta1 - theta2))/4 + (L2*L4*m5*theta1_ddot*cos(theta1 - theta2))/4 - (L2^2*m3*theta1_dot*theta2_dot*sin(theta2 - theta1 + theta3))/4 - (L3^2*m4*theta1_dot*theta2_dot*sin(theta2 - theta1 + theta3))/2 - (L3^2*m4*theta1_dot*theta3_dot*sin(theta2 - theta1 + theta3))/2 + (L3^2*m4*theta2_dot*theta3_dot*sin(theta2 - theta1 + theta3))/2 - (L4^2*m5*theta1_dot*theta2_dot*sin(theta2 - theta1 + theta3))/2 - (L4^2*m5*theta1_dot*theta3_dot*sin(theta2 - theta1 + theta3))/2 + (L4^2*m5*theta2_dot*theta3_dot*sin(theta2 - theta1 + theta3))/2 - (L2*L3*m4*theta1_dot^2*sin(theta1 + theta2))/4 - (L2*L4*m5*theta1_dot^2*sin(theta1 + theta2))/4 + (d2*d3*m3*theta1_dot^2*sin(theta1 + 2*theta2 + theta3))/2 + (d2*d4*m4*theta1_dot^2*sin(theta1 + 2*theta2 + theta3))/2 + d3*d4*m4*theta1_dot^2*sin(theta1 + theta2 + 2*theta3) + (L2*L3*m4*theta2_ddot*cos(theta1 + theta2 + theta3))/4 + (L2*L4*m5*theta2_ddot*cos(theta1 + theta2 + theta3))/4 + (L3*L4*m5*theta1_ddot*cos(theta1 + theta2 + theta3))/4 + (L3*L4*m5*theta2_ddot*cos(theta1 + theta2 + theta3))/2 + (L3*L4*m5*theta3_ddot*cos(theta1 + theta2 + theta3))/2 + (L2*d2*m3*theta1_dot^2*cos(theta1 + theta2))/4 + (3*L2*d3*m3*theta1_dot^2*cos(theta1 + theta3))/4 + (L3*d2*m4*theta1_dot^2*cos(theta1 + theta2))/4 + (L2*d4*m4*theta1_dot^2*cos(theta1 + theta3))/2 + (L3*d3*m4*theta1_dot^2*cos(theta1 + theta3))/4 + (L4*d2*m5*theta1_dot^2*cos(theta1 + theta2))/4 + (L4*d3*m5*theta1_dot^2*cos(theta1 + theta3))/4 - (L2*L3*m4*theta1_dot*theta2_dot*sin(theta1 + theta2))/4 - (L2*L4*m5*theta1_dot*theta2_dot*sin(theta1 + theta2))/4 + (L2*d2*m3*theta1_dot*theta2_dot*cos(theta1 + theta2))/4 - (L2*d3*m3*theta1_dot*theta2_dot*cos(theta1 + theta3))/4 + (L3*d2*m4*theta1_dot*theta2_dot*cos(theta1 + theta2))/4 - (L3*d3*m4*theta1_dot*theta2_dot*cos(theta1 + theta3))/4 + (L4*d2*m5*theta1_dot*theta2_dot*cos(theta1 + theta2))/4 + L2*d4*m4*theta1_dot*theta2_dot*cos(theta2 + theta3) + L2*d4*m5*theta1_dot*theta2_dot*cos(theta2 + theta3) - (L4*d3*m5*theta1_dot*theta2_dot*cos(theta1 + theta3))/4 + L2*d2*m3*theta1_dot*theta2_dot*cos(theta3) + L2*d2*m4*theta1_dot*theta2_dot*cos(theta3) + L2*d2*m5*theta1_dot*theta2_dot*cos(theta3) + L3*d2*m4*theta1_dot*theta2_dot*cos(theta3) - L3*d3*m4*theta1_dot*theta2_dot*cos(theta2) + L3*d2*m5*theta1_dot*theta2_dot*cos(theta3) - L3*d3*m5*theta1_dot*theta2_dot*cos(theta2) + L4*d2*m5*theta1_dot*theta2_dot*cos(theta3) - L4*d3*m5*theta1_dot*theta2_dot*cos(theta2) + L2*d3*m3*theta1_dot*theta2_dot*cos(theta1 + 2*theta2 + 2*theta3) + L2*d4*m4*theta1_dot*theta2_dot*cos(theta1 + 2*theta2 + 2*theta3) + (L2*L3*m4*theta1_dot*theta2_dot*sin(theta1 - theta2))/4 + (L2*L4*m5*theta1_dot*theta2_dot*sin(theta1 - theta2))/4 - (L2*d2*m3*theta1_dot*theta2_dot*cos(theta1 - theta2))/4 + (L2*d3*m3*theta1_dot*theta2_dot*cos(theta1 - theta3))/4 - (L3*d2*m4*theta1_dot*theta2_dot*cos(theta1 - theta2))/4 + (L3*d3*m4*theta1_dot*theta2_dot*cos(theta1 - theta3))/4 - (L4*d2*m5*theta1_dot*theta2_dot*cos(theta1 - theta2))/4 + (L4*d3*m5*theta1_dot*theta2_dot*cos(theta1 - theta3))/4 - (L2*L3*m4*theta1_dot*theta2_dot*sin(theta1 + theta2 + theta3))/4 - (L2*L4*m5*theta1_dot*theta2_dot*sin(theta1 + theta2 + theta3))/4 - (L3*L4*m5*theta1_dot*theta2_dot*sin(theta1 + theta2 + theta3))/2 - (L3*L4*m5*theta1_dot*theta3_dot*sin(theta1 + theta2 + theta3))/2 - (L3*L4*m5*theta2_dot*theta3_dot*sin(theta1 + theta2 + theta3))/2 - (L2*L3*m4*theta1_dot*theta2_dot*sin(2*theta2 + 2*theta3))/2 - (L2*L4*m5*theta1_dot*theta2_dot*sin(2*theta2 + 2*theta3))/2 - (L2*L3*m4*theta1_dot*theta2_dot*sin(theta2 - theta1 + theta3))/4 - (L2*L4*m5*theta1_dot*theta2_dot*sin(theta2 - theta1 + theta3))/4 - (L3*L4*m5*theta1_dot*theta2_dot*sin(theta2 - theta1 + theta3))/2 - (L3*L4*m5*theta1_dot*theta3_dot*sin(theta2 - theta1 + theta3))/2 + (L3*L4*m5*theta2_dot*theta3_dot*sin(theta2 - theta1 + theta3))/2;
    M = [2*I1 + 2*I2 + 2*I3 + 2*I4 + 2*I5 + (5*L2^2*m3)/8 + (L2^2*m4)/2 + (L2^2*m5)/2 + (5*L3^2*m4)/8 + (L3^2*m5)/2 + (5*L4^2*m5)/8 + (d2^2*m2)/2 + d2^2*m3 + d2^2*m4 + 2*d3^2*m3 + d2^2*m5 + d3^2*m4 + d3^2*m5 + 2*d4^2*m4 + d4^2*m5 + d3^2*m3*cos(theta1 + theta2 + 2*theta3) + d3^2*m3*cos(theta1 + theta2) + L3*L4*m5 + (L2^2*m3*cos(2*theta2))/2 + (L2^2*m4*cos(2*theta2))/2 + (L2^2*m5*cos(2*theta2))/2 + 2*d4^2*m4*cos(theta1 + theta2 + theta3) + (d2^2*m2*cos(2*theta2))/2 + (L2^2*m3*cos(2*theta2 + 2*theta3))/8 + (5*L3^2*m4*cos(2*theta2 + 2*theta3))/8 + (L3^2*m5*cos(2*theta2 + 2*theta3))/2 + (5*L4^2*m5*cos(2*theta2 + 2*theta3))/8 - L2*d3*m3*sin(theta1 + 2*theta2 + theta3) - L2*d4*m4*sin(theta1 + 2*theta2 + theta3) + d2*d3*m3*cos(theta1 + 2*theta2 + theta3) + d2*d4*m4*cos(theta1 + 2*theta2 + theta3) + d3*d4*m4*cos(theta1 + theta2 + 2*theta3) - L2*d3*m3*sin(theta1 + theta3) - L2*d4*m4*sin(theta1 + theta3) + L2*L3*m4*cos(theta3) + L2*L3*m5*cos(theta3) + L2*L4*m5*cos(theta3) + d2*d3*m3*cos(theta1 + theta3) + d2*d4*m4*cos(theta1 + theta3) + d3*d4*m4*cos(theta1 + theta2) + (L2*d2*m3*sin(theta3))/2 + (L2*d3*m3*sin(theta2))/2 + (L3*d2*m4*sin(theta3))/2 + (L3*d3*m4*sin(theta2))/2 - L3*d4*m4*sin(theta1) + (L4*d2*m5*sin(theta3))/2 + (L4*d3*m5*sin(theta2))/2 - L3*d4*m4*sin(theta1 + 2*theta2 + 2*theta3) + 2*d2*d4*m4*cos(theta2) + 2*d2*d4*m5*cos(theta2) + 2*d3*d4*m4*cos(theta3) + 2*d3*d4*m5*cos(theta3) + L2*L3*m4*cos(2*theta2 + theta3) + L2*L3*m5*cos(2*theta2 + theta3) + L2*L4*m5*cos(2*theta2 + theta3) - (L2*d2*m3*sin(2*theta2 + theta3))/2 - (L2*d3*m3*sin(theta2 + 2*theta3))/2 - (L3*d2*m4*sin(2*theta2 + theta3))/2 - (L3*d3*m4*sin(theta2 + 2*theta3))/2 - (L4*d2*m5*sin(2*theta2 + theta3))/2 - (L4*d3*m5*sin(theta2 + 2*theta3))/2 + 2*d2*d3*m3*cos(theta2 - theta3) + 2*d2*d3*m4*cos(theta2 - theta3) + 2*d2*d3*m5*cos(theta2 - theta3) + L3*L4*m5*cos(2*theta2 + 2*theta3), (L2^2*m3*cos(theta1 + theta2))/4 - (L3^2*m4)/4 - (L4^2*m5)/4 - (L2^2*m3)/4 + (d2^2*m2*cos(theta1 + theta2))/2 - (L2*L3*m4)/4 - (L2*L4*m5)/4 - (L3*L4*m5)/4 + (L2^2*m3*cos(theta1 - theta2))/4 + (L3^2*m4*cos(theta1 + theta2 + theta3))/4 + (L4^2*m5*cos(theta1 + theta2 + theta3))/4 + (d2^2*m2*cos(theta1 - theta2))/2 - (L2^2*m3*cos(2*theta2 + 2*theta3))/4 - (L3^2*m4*cos(2*theta2 + 2*theta3))/4 - (L4^2*m5*cos(2*theta2 + 2*theta3))/4 + (L3^2*m4*cos(theta2 - theta1 + theta3))/4 + (L4^2*m5*cos(theta2 - theta1 + theta3))/4 + (L2*L3*m4*cos(theta1 + theta2))/4 + (L2*L4*m5*cos(theta1 + theta2))/4 + (L2*d2*m3*sin(theta1 + theta2))/4 + (L2*d3*m3*sin(theta1 + theta3))/4 + (L3*d2*m4*sin(theta1 + theta2))/4 - (L2*d3*m3*sin(theta2 + theta3))/2 + (L3*d3*m4*sin(theta1 + theta3))/4 + (L4*d2*m5*sin(theta1 + theta2))/4 - L2*d4*m4*sin(theta2 + theta3) - L2*d4*m5*sin(theta2 + theta3) - (3*L3*d4*m4*sin(theta2 + theta3))/2 + (L4*d3*m5*sin(theta1 + theta3))/4 - L3*d4*m5*sin(theta2 + theta3) - L4*d4*m5*sin(theta2 + theta3) + (L2*d3*m3*sin(theta1))/2 - L2*d2*m3*sin(theta3) - L2*d3*m3*sin(theta2) - L2*d2*m4*sin(theta3) - L2*d3*m4*sin(theta2) + (L2*d4*m4*sin(theta1))/2 - L2*d2*m5*sin(theta3) - L2*d3*m5*sin(theta2) - L3*d2*m4*sin(theta3) - L3*d3*m4*sin(theta2) + L3*d4*m4*sin(theta1) - L3*d2*m5*sin(theta3) - L3*d3*m5*sin(theta2) - L4*d2*m5*sin(theta3) - L4*d3*m5*sin(theta2) + (L4*d4*m5*sin(theta1))/2 - (L2*d3*m3*sin(theta1 + 2*theta2 + 2*theta3))/2 - (L2*d4*m4*sin(theta1 + 2*theta2 + 2*theta3))/2 - (L3*d4*m4*sin(theta1 + 2*theta2 + 2*theta3))/2 + (L2*L3*m4*cos(theta1 - theta2))/4 + (L2*L4*m5*cos(theta1 - theta2))/4 + (L3*L4*m5*cos(theta1 + theta2 + theta3))/4 + (L2*d2*m3*sin(theta1 - theta2))/4 + (L2*d3*m3*sin(theta1 - theta3))/4 + (L3*d2*m4*sin(theta1 - theta2))/4 + (L3*d3*m4*sin(theta1 - theta3))/4 + (L4*d2*m5*sin(theta1 - theta2))/4 + (L4*d3*m5*sin(theta1 - theta3))/4 - (L2*L3*m4*cos(2*theta2 + 2*theta3))/4 - (L2*L4*m5*cos(2*theta2 + 2*theta3))/4 - (L3*L4*m5*cos(2*theta2 + 2*theta3))/4 + (L3*L4*m5*cos(theta2 - theta1 + theta3))/4, (L2^2*m3*cos(theta1 + theta2))/4 - (L4^2*m5)/4 - (L3^2*m4)/4 - (L3*L4*m5)/4 + (L2^2*m3*cos(theta1 - theta2))/4 + (L3^2*m4*cos(theta1 + theta2 + theta3))/4 + (L4^2*m5*cos(theta1 + theta2 + theta3))/4 - (L3^2*m4*cos(2*theta2 + 2*theta3))/4 - (L4^2*m5*cos(2*theta2 + 2*theta3))/4 + (L3^2*m4*cos(theta2 - theta1 + theta3))/4 + (L4^2*m5*cos(theta2 - theta1 + theta3))/4 + (L2*L3*m4*cos(theta1 + theta2))/4 + (L2*L4*m5*cos(theta1 + theta2))/4 + (L2*d2*m3*sin(theta1 + theta2))/4 + (L2*d3*m3*sin(theta1 + theta3))/4 + (L3*d2*m4*sin(theta1 + theta2))/4 - (L2*d3*m3*sin(theta2 + theta3))/2 + (L3*d3*m4*sin(theta1 + theta3))/4 + (L4*d2*m5*sin(theta1 + theta2))/4 - (3*L3*d4*m4*sin(theta2 + theta3))/2 + (L4*d3*m5*sin(theta1 + theta3))/4 - L3*d4*m5*sin(theta2 + theta3) - L4*d4*m5*sin(theta2 + theta3) - L3*d2*m4*sin(theta3) - L3*d3*m4*sin(theta2) + L3*d4*m4*sin(theta1) - L3*d2*m5*sin(theta3) - L3*d3*m5*sin(theta2) - L4*d2*m5*sin(theta3) - L4*d3*m5*sin(theta2) + (L4*d4*m5*sin(theta1))/2 - (L3*d4*m4*sin(theta1 + 2*theta2 + 2*theta3))/2 + (L2*L3*m4*cos(theta1 - theta2))/4 + (L2*L4*m5*cos(theta1 - theta2))/4 + (L3*L4*m5*cos(theta1 + theta2 + theta3))/4 + (L2*d2*m3*sin(theta1 - theta2))/4 + (L2*d3*m3*sin(theta1 - theta3))/4 + (L3*d2*m4*sin(theta1 - theta2))/4 + (L3*d3*m4*sin(theta1 - theta3))/4 + (L4*d2*m5*sin(theta1 - theta2))/4 + (L4*d3*m5*sin(theta1 - theta3))/4 - (L3*L4*m5*cos(2*theta2 + 2*theta3))/4 + (L3*L4*m5*cos(theta2 - theta1 + theta3))/4];
    (L2^2*m3*cos(theta1 + theta2))/4 - (L3^2*m4)/4 - (L4^2*m5)/4 - (L2^2*m3)/4 + (d2^2*m2*cos(theta1 + theta2))/2 - (L2*L3*m4)/4 - (L2*L4*m5)/4 - (L3*L4*m5)/4 + (L2^2*m3*cos(theta1 - theta2))/4 + (L3^2*m4*cos(theta1 + theta2 + theta3))/4 + (L4^2*m5*cos(theta1 + theta2 + theta3))/4 + (d2^2*m2*cos(theta1 - theta2))/2 - (L2^2*m3*cos(2*theta2 + 2*theta3))/4 - (L3^2*m4*cos(2*theta2 + 2*theta3))/4 - (L4^2*m5*cos(2*theta2 + 2*theta3))/4 + (L3^2*m4*cos(theta2 - theta1 + theta3))/4 + (L4^2*m5*cos(theta2 - theta1 + theta3))/4 + (L2*L3*m4*cos(theta1 + theta2))/4 + (L2*L4*m5*cos(theta1 + theta2))/4 + (L2*d2*m3*sin(theta1 + theta2))/4 + (L2*d3*m3*sin(theta1 + theta3))/4 + (L3*d2*m4*sin(theta1 + theta2))/4 - (L2*d3*m3*sin(theta2 + theta3))/2 + (L3*d3*m4*sin(theta1 + theta3))/4 + (L4*d2*m5*sin(theta1 + theta2))/4 - L2*d4*m4*sin(theta2 + theta3) - L2*d4*m5*sin(theta2 + theta3) - (3*L3*d4*m4*sin(theta2 + theta3))/2 + (L4*d3*m5*sin(theta1 + theta3))/4 - L3*d4*m5*sin(theta2 + theta3) - L4*d4*m5*sin(theta2 + theta3) + (L2*d3*m3*sin(theta1))/2 - L2*d2*m3*sin(theta3) - L2*d3*m3*sin(theta2) - L2*d2*m4*sin(theta3) - L2*d3*m4*sin(theta2) + (L2*d4*m4*sin(theta1))/2 - L2*d2*m5*sin(theta3) - L2*d3*m5*sin(theta2) - L3*d2*m4*sin(theta3) - L3*d3*m4*sin(theta2) + L3*d4*m4*sin(theta1) - L3*d2*m5*sin(theta3) - L3*d3*m5*sin(theta2) - L4*d2*m5*sin(theta3) - L4*d3*m5*sin(theta2) + (L4*d4*m5*sin(theta1))/2 - (L2*d3*m3*sin(theta1 + 2*theta2 + 2*theta3))/2 - (L2*d4*m4*sin(theta1 + 2*theta2 + 2*theta3))/2 - (L3*d4*m4*sin(theta1 + 2*theta2 + 2*theta3))/2 + (L2*L3*m4*cos(theta1 - theta2))/4 + (L2*L4*m5*cos(theta1 - theta2))/4 + (L3*L4*m5*cos(theta1 + theta2 + theta3))/4 + (L2*d2*m3*sin(theta1 - theta2))/4 + (L2*d3*m3*sin(theta1 - theta3))/4 + (L3*d2*m4*sin(theta1 - theta2))/4 + (L3*d3*m4*sin(theta1 - theta3))/4 + (L4*d2*m5*sin(theta1 - theta2))/4 + (L4*d3*m5*sin(theta1 - theta3))/4 - (L2*L3*m4*cos(2*theta2 + 2*theta3))/4 - (L2*L4*m5*cos(2*theta2 + 2*theta3))/4 - (L3*L4*m5*cos(2*theta2 + 2*theta3))/4 + (L3*L4*m5*cos(theta2 - theta1 + theta3))/4,                                                                                                                                                                                                                                                                                                                                                                                                                                                                                                                                                                                                                                                                                                                                                                                                                                                                                                                                                                                                                                                                                                                                                                                                                                                                                                                                                              2*I2 + 2*I3 + 2*I4 + 2*I5 + (5*L2^2*m3)/4 + L2^2*m4 + L2^2*m5 + (5*L3^2*m4)/4 + L3^2*m5 + (5*L4^2*m5)/4 + d2^2*m2 + 2*L2*L3*m4 + 2*L2*L3*m5 + 2*L2*L4*m5 + 2*L3*L4*m5 - L2^2*m3*cos(theta2)*sin(theta1)*sin(theta3) - L2^2*m3*cos(theta3)*sin(theta1)*sin(theta2) - L3^2*m4*cos(theta2)*sin(theta1)*sin(theta3) - L3^2*m4*cos(theta3)*sin(theta1)*sin(theta2) - L4^2*m5*cos(theta2)*sin(theta1)*sin(theta3) - L4^2*m5*cos(theta3)*sin(theta1)*sin(theta2) - L2*L3*m4*cos(theta2)*sin(theta1)*sin(theta3) - L2*L3*m4*cos(theta3)*sin(theta1)*sin(theta2) - L2*L4*m5*cos(theta2)*sin(theta1)*sin(theta3) - L2*L4*m5*cos(theta3)*sin(theta1)*sin(theta2) - L3*L4*m5*cos(theta2)*sin(theta1)*sin(theta3) - L3*L4*m5*cos(theta3)*sin(theta1)*sin(theta2),                                                                                                                                                                                                                                                                                                                                                                                                                                                                                                                                                                                                                                                                                                                                                                        2*I3 + 2*I4 + 2*I5 + (L2^2*m3)/4 + (5*L3^2*m4)/4 + L3^2*m5 + (5*L4^2*m5)/4 + L2*L3*m4 + L2*L3*m5 + L2*L4*m5 + 2*L3*L4*m5 - (L2^2*m3*cos(theta2)*sin(theta1)*sin(theta3))/2 - (L2^2*m3*cos(theta3)*sin(theta1)*sin(theta2))/2 - L3^2*m4*cos(theta2)*sin(theta1)*sin(theta3) - L3^2*m4*cos(theta3)*sin(theta1)*sin(theta2) - L4^2*m5*cos(theta2)*sin(theta1)*sin(theta3) - L4^2*m5*cos(theta3)*sin(theta1)*sin(theta2) - (L2*L3*m4*cos(theta2)*sin(theta1)*sin(theta3))/2 - (L2*L3*m4*cos(theta3)*sin(theta1)*sin(theta2))/2 - (L2*L4*m5*cos(theta2)*sin(theta1)*sin(theta3))/2 - (L2*L4*m5*cos(theta3)*sin(theta1)*sin(theta2))/2 - L3*L4*m5*cos(theta2)*sin(theta1)*sin(theta3) - L3*L4*m5*cos(theta3)*sin(theta1)*sin(theta2);
    G =[
 
 - g*m3*(d2*sin(theta1) + 2*d3*sin(theta1) - (L2*(cos(theta1)*sin(theta2)*sin(theta3) - cos(theta1)*cos(theta2)*cos(theta3)))/2 + L2*cos(theta1)*cos(theta2)) - g*m2*(d2*sin(theta1) + d2*cos(theta1)*sin(theta2)) - g*m5*(d2*sin(theta1) + d3*sin(theta1) + d4*sin(theta1) - L3*(cos(theta1)*sin(theta2)*sin(theta3) - cos(theta1)*cos(theta2)*cos(theta3)) - (3*L4*(cos(theta1)*sin(theta2)*sin(theta3) - cos(theta1)*cos(theta2)*cos(theta3)))/2 + L2*cos(theta1)*cos(theta2)) - g*m4*(d2*sin(theta1) + d3*sin(theta1) + 2*d4*sin(theta1) - (3*L3*(cos(theta1)*sin(theta2)*sin(theta3) - cos(theta1)*cos(theta2)*cos(theta3)))/2 + L2*cos(theta1)*cos(theta2));
                                                                                                                                                                                                                                                                                                                                                                                                                              (g*sin(theta1)*(2*L2*m3*sin(theta2) + 2*L2*m4*sin(theta2) + 2*L2*m5*sin(theta2) - 2*d2*m2*cos(theta2) + L2*m3*sin(theta2 + theta3) + 3*L3*m4*sin(theta2 + theta3) + 2*L3*m5*sin(theta2 + theta3) + 3*L4*m5*sin(theta2 + theta3)))/2;
                                                                                                                                                                                                                                                                                                                                                                                                                                                                                                                                                                                     (g*sin(theta2 + theta3)*sin(theta1)*(L2*m3 + 3*L3*m4 + 2*L3*m5 + 3*L4*m5))/2];
    V =[
 
 (L2^2*m3*theta2_dot^2*sin(theta1 - theta2))/4 - (d2^2*m2*theta2_dot^2*sin(theta1 + theta2))/2 - (d3^2*m3*theta1_dot^2*sin(theta1 + theta2))/2 - (L2^2*m3*theta2_dot^2*sin(theta1 + theta2))/4 + (L2^2*m3*theta2_dot^2*sin(theta1 + theta2 + theta3))/4 + (d2^2*m2*theta2_dot^2*sin(theta1 - theta2))/2 - d4^2*m4*theta1_dot^2*sin(theta1 + theta2 + theta3) + (L2^2*m3*theta2_dot^2*sin(2*theta2 + 2*theta3))/2 + (L3^2*m4*theta2_dot^2*sin(2*theta2 + 2*theta3))/2 + (L3^2*m4*theta3_dot^2*sin(2*theta2 + 2*theta3))/2 + (L4^2*m5*theta2_dot^2*sin(2*theta2 + 2*theta3))/2 + (L4^2*m5*theta3_dot^2*sin(2*theta2 + 2*theta3))/2 + (L2^2*m3*theta2_dot^2*sin(theta2 - theta1 + theta3))/4 - (d3^2*m3*theta1_dot^2*sin(theta1 + theta2 + 2*theta3))/2 - d3^2*m3*theta1_dot*theta2_dot*sin(theta1 + theta2 + 2*theta3) - 2*d3^2*m3*theta1_dot*theta3_dot*sin(theta1 + theta2 + 2*theta3) - (L2^2*m3*theta2_dot*theta3_dot*sin(theta1 + theta2))/4 - (d2*d3*m3*theta1_dot^2*sin(theta1 + theta3))/2 - (d2*d4*m4*theta1_dot^2*sin(theta1 + theta3))/2 - (d3*d4*m4*theta1_dot^2*sin(theta1 + theta2))/2 - L2*d3*m3*theta2_dot^2*cos(theta2) - L2*d3*m4*theta2_dot^2*cos(theta2) - (L3*d4*m4*theta1_dot^2*cos(theta1))/2 - L2*d3*m5*theta2_dot^2*cos(theta2) - L3*d3*m4*theta2_dot^2*cos(theta2) - L3*d2*m4*theta3_dot^2*cos(theta3) - L3*d3*m5*theta2_dot^2*cos(theta2) - L3*d2*m5*theta3_dot^2*cos(theta3) - L4*d3*m5*theta2_dot^2*cos(theta2) - L4*d2*m5*theta3_dot^2*cos(theta3) - L2*d3*m3*theta2_dot^2*cos(theta1 + 2*theta2 + 2*theta3) - L2*d4*m4*theta2_dot^2*cos(theta1 + 2*theta2 + 2*theta3) - (L3*d4*m4*theta1_dot^2*cos(theta1 + 2*theta2 + 2*theta3))/2 - L3*d4*m4*theta2_dot^2*cos(theta1 + 2*theta2 + 2*theta3) - L3*d4*m4*theta3_dot^2*cos(theta1 + 2*theta2 + 2*theta3) - d3^2*m3*theta1_dot*theta2_dot*sin(theta1 + theta2) + (L2*L3*m4*theta2_dot^2*sin(theta1 - theta2))/4 + (L2*L4*m5*theta2_dot^2*sin(theta1 - theta2))/4 - (L2*d2*m3*theta2_dot^2*cos(theta1 - theta2))/4 - (L3*d2*m4*theta2_dot^2*cos(theta1 - theta2))/4 - (L2*d3*m3*theta3_dot^2*cos(theta1 - theta3))/4 - (L4*d2*m5*theta2_dot^2*cos(theta1 - theta2))/4 - (L3*d3*m4*theta3_dot^2*cos(theta1 - theta3))/4 - (L4*d3*m5*theta3_dot^2*cos(theta1 - theta3))/4 + (L2*L3*m4*theta2_dot^2*sin(theta1 + theta2 + theta3))/4 + (L2*L4*m5*theta2_dot^2*sin(theta1 + theta2 + theta3))/4 + (L2^2*m3*theta2_dot*theta3_dot*sin(theta1 - theta2))/4 + (L2^2*m3*theta2_dot*theta3_dot*sin(theta1 + theta2 + theta3))/4 - L2^2*m3*theta1_dot*theta2_dot*sin(2*theta2) - L2^2*m4*theta1_dot*theta2_dot*sin(2*theta2) - L2^2*m5*theta1_dot*theta2_dot*sin(2*theta2) - 2*d4^2*m4*theta1_dot*theta2_dot*sin(theta1 + theta2 + theta3) - 2*d4^2*m4*theta1_dot*theta3_dot*sin(theta1 + theta2 + theta3) + (L2*L3*m4*theta2_dot^2*sin(2*theta2 + 2*theta3))/2 + (L2*L4*m5*theta2_dot^2*sin(2*theta2 + 2*theta3))/2 + (L3*L4*m5*theta2_dot^2*sin(2*theta2 + 2*theta3))/2 + (L3*L4*m5*theta3_dot^2*sin(2*theta2 + 2*theta3))/2 - d2^2*m2*theta1_dot*theta2_dot*sin(2*theta2) + (L2*L3*m4*theta2_dot^2*sin(theta2 - theta1 + theta3))/4 + (L2*L4*m5*theta2_dot^2*sin(theta2 - theta1 + theta3))/4 - (L2*d3*m3*theta1_dot^2*cos(theta1 + 2*theta2 + theta3))/2 - (L2*d4*m4*theta1_dot^2*cos(theta1 + 2*theta2 + theta3))/2 - (L2^2*m3*theta1_dot*theta2_dot*sin(2*theta2 + 2*theta3))/4 - (L2^2*m3*theta1_dot*theta3_dot*sin(2*theta2 + 2*theta3))/4 + (L2^2*m3*theta2_dot*theta3_dot*sin(2*theta2 + 2*theta3))/2 - (5*L3^2*m4*theta1_dot*theta2_dot*sin(2*theta2 + 2*theta3))/4 - (5*L3^2*m4*theta1_dot*theta3_dot*sin(2*theta2 + 2*theta3))/4 - L3^2*m5*theta1_dot*theta2_dot*sin(2*theta2 + 2*theta3) + L3^2*m4*theta2_dot*theta3_dot*sin(2*theta2 + 2*theta3) - L3^2*m5*theta1_dot*theta3_dot*sin(2*theta2 + 2*theta3) - (5*L4^2*m5*theta1_dot*theta2_dot*sin(2*theta2 + 2*theta3))/4 - (5*L4^2*m5*theta1_dot*theta3_dot*sin(2*theta2 + 2*theta3))/4 + L4^2*m5*theta2_dot*theta3_dot*sin(2*theta2 + 2*theta3) + (L2^2*m3*theta2_dot*theta3_dot*sin(theta2 - theta1 + theta3))/4 - (L2*L3*m4*theta2_dot^2*sin(theta1 + theta2))/4 - (L2*L4*m5*theta2_dot^2*sin(theta1 + theta2))/4 - (d2*d3*m3*theta1_dot^2*sin(theta1 + 2*theta2 + theta3))/2 - (d2*d4*m4*theta1_dot^2*sin(theta1 + 2*theta2 + theta3))/2 - (d3*d4*m4*theta1_dot^2*sin(theta1 + theta2 + 2*theta3))/2 + (L2*d2*m3*theta2_dot^2*cos(theta1 + theta2))/4 - (L2*d3*m3*theta1_dot^2*cos(theta1 + theta3))/2 + (L3*d2*m4*theta2_dot^2*cos(theta1 + theta2))/4 - (L2*d3*m3*theta2_dot^2*cos(theta2 + theta3))/2 + (L2*d3*m3*theta3_dot^2*cos(theta1 + theta3))/4 - (L2*d4*m4*theta1_dot^2*cos(theta1 + theta3))/2 - (L2*d3*m3*theta3_dot^2*cos(theta2 + theta3))/2 + (L4*d2*m5*theta2_dot^2*cos(theta1 + theta2))/4 - L2*d4*m4*theta2_dot^2*cos(theta2 + theta3) + (L3*d3*m4*theta3_dot^2*cos(theta1 + theta3))/4 - L2*d4*m5*theta2_dot^2*cos(theta2 + theta3) - (3*L3*d4*m4*theta2_dot^2*cos(theta2 + theta3))/2 - (3*L3*d4*m4*theta3_dot^2*cos(theta2 + theta3))/2 - L3*d4*m5*theta2_dot^2*cos(theta2 + theta3) + (L4*d3*m5*theta3_dot^2*cos(theta1 + theta3))/4 - L3*d4*m5*theta3_dot^2*cos(theta2 + theta3) - L4*d4*m5*theta2_dot^2*cos(theta2 + theta3) - L4*d4*m5*theta3_dot^2*cos(theta2 + theta3) - (L2*L3*m4*theta2_dot*theta3_dot*sin(theta1 + theta2))/4 - (L2*L4*m5*theta2_dot*theta3_dot*sin(theta1 + theta2))/4 - 2*d2*d3*m3*theta1_dot*theta2_dot*sin(theta1 + 2*theta2 + theta3) - d2*d3*m3*theta1_dot*theta3_dot*sin(theta1 + 2*theta2 + theta3) - 2*d2*d4*m4*theta1_dot*theta2_dot*sin(theta1 + 2*theta2 + theta3) - d2*d4*m4*theta1_dot*theta3_dot*sin(theta1 + 2*theta2 + theta3) - d3*d4*m4*theta1_dot*theta2_dot*sin(theta1 + theta2 + 2*theta3) - 2*d3*d4*m4*theta1_dot*theta3_dot*sin(theta1 + theta2 + 2*theta3) + (L2*d2*m3*theta2_dot*theta3_dot*cos(theta1 + theta2))/4 - L2*d3*m3*theta1_dot*theta3_dot*cos(theta1 + theta3) + (L2*d3*m3*theta2_dot*theta3_dot*cos(theta1 + theta3))/4 + (L3*d2*m4*theta2_dot*theta3_dot*cos(theta1 + theta2))/4 - L2*d3*m3*theta2_dot*theta3_dot*cos(theta2 + theta3) - L2*d4*m4*theta1_dot*theta3_dot*cos(theta1 + theta3) + (L3*d3*m4*theta2_dot*theta3_dot*cos(theta1 + theta3))/4 + (L4*d2*m5*theta2_dot*theta3_dot*cos(theta1 + theta2))/4 - L2*d4*m4*theta2_dot*theta3_dot*cos(theta2 + theta3) - L2*d4*m5*theta2_dot*theta3_dot*cos(theta2 + theta3) - 3*L3*d4*m4*theta2_dot*theta3_dot*cos(theta2 + theta3) + (L4*d3*m5*theta2_dot*theta3_dot*cos(theta1 + theta3))/4 - 2*L3*d4*m5*theta2_dot*theta3_dot*cos(theta2 + theta3) - 2*L4*d4*m5*theta2_dot*theta3_dot*cos(theta2 + theta3) - L2*L3*m4*theta1_dot*theta3_dot*sin(theta3) - L2*L3*m5*theta1_dot*theta3_dot*sin(theta3) - L2*L4*m5*theta1_dot*theta3_dot*sin(theta3) - d2*d3*m3*theta1_dot*theta3_dot*sin(theta1 + theta3) - d3*d4*m4*theta1_dot*theta2_dot*sin(theta1 + theta2) - d2*d4*m4*theta1_dot*theta3_dot*sin(theta1 + theta3) + (L2*d3*m3*theta1_dot*theta2_dot*cos(theta2))/2 + (L2*d2*m3*theta1_dot*theta3_dot*cos(theta3))/2 - L2*d2*m3*theta2_dot*theta3_dot*cos(theta3) + (L3*d3*m4*theta1_dot*theta2_dot*cos(theta2))/2 - L2*d2*m4*theta2_dot*theta3_dot*cos(theta3) + (L3*d2*m4*theta1_dot*theta3_dot*cos(theta3))/2 - L2*d2*m5*theta2_dot*theta3_dot*cos(theta3) - L3*d2*m4*theta2_dot*theta3_dot*cos(theta3) - L3*d3*m4*theta2_dot*theta3_dot*cos(theta2) + (L4*d3*m5*theta1_dot*theta2_dot*cos(theta2))/2 - L3*d2*m5*theta2_dot*theta3_dot*cos(theta3) - L3*d3*m5*theta2_dot*theta3_dot*cos(theta2) + (L4*d2*m5*theta1_dot*theta3_dot*cos(theta3))/2 - L4*d2*m5*theta2_dot*theta3_dot*cos(theta3) - L4*d3*m5*theta2_dot*theta3_dot*cos(theta2) - L2*d3*m3*theta2_dot*theta3_dot*cos(theta1 + 2*theta2 + 2*theta3) - 2*L3*d4*m4*theta1_dot*theta2_dot*cos(theta1 + 2*theta2 + 2*theta3) - L2*d4*m4*theta2_dot*theta3_dot*cos(theta1 + 2*theta2 + 2*theta3) - 2*L3*d4*m4*theta1_dot*theta3_dot*cos(theta1 + 2*theta2 + 2*theta3) - 2*L3*d4*m4*theta2_dot*theta3_dot*cos(theta1 + 2*theta2 + 2*theta3) - 2*d2*d4*m4*theta1_dot*theta2_dot*sin(theta2) - 2*d2*d4*m5*theta1_dot*theta2_dot*sin(theta2) - 2*d3*d4*m4*theta1_dot*theta3_dot*sin(theta3) - 2*d3*d4*m5*theta1_dot*theta3_dot*sin(theta3) + (L2*L3*m4*theta2_dot*theta3_dot*sin(theta1 - theta2))/4 - 2*L2*L3*m4*theta1_dot*theta2_dot*sin(2*theta2 + theta3) - L2*L3*m4*theta1_dot*theta3_dot*sin(2*theta2 + theta3) - 2*L2*L3*m5*theta1_dot*theta2_dot*sin(2*theta2 + theta3) + (L2*L4*m5*theta2_dot*theta3_dot*sin(theta1 - theta2))/4 - L2*L3*m5*theta1_dot*theta3_dot*sin(2*theta2 + theta3) - 2*L2*L4*m5*theta1_dot*theta2_dot*sin(2*theta2 + theta3) - L2*L4*m5*theta1_dot*theta3_dot*sin(2*theta2 + theta3) - (L2*d2*m3*theta2_dot*theta3_dot*cos(theta1 - theta2))/4 - L2*d2*m3*theta1_dot*theta2_dot*cos(2*theta2 + theta3) - (L2*d2*m3*theta1_dot*theta3_dot*cos(2*theta2 + theta3))/2 - (L2*d3*m3*theta1_dot*theta2_dot*cos(theta2 + 2*theta3))/2 - (L2*d3*m3*theta2_dot*theta3_dot*cos(theta1 - theta3))/4 - (L3*d2*m4*theta2_dot*theta3_dot*cos(theta1 - theta2))/4 - L2*d3*m3*theta1_dot*theta3_dot*cos(theta2 + 2*theta3) - L3*d2*m4*theta1_dot*theta2_dot*cos(2*theta2 + theta3) - (L3*d2*m4*theta1_dot*theta3_dot*cos(2*theta2 + theta3))/2 - (L3*d3*m4*theta1_dot*theta2_dot*cos(theta2 + 2*theta3))/2 - (L3*d3*m4*theta2_dot*theta3_dot*cos(theta1 - theta3))/4 - (L4*d2*m5*theta2_dot*theta3_dot*cos(theta1 - theta2))/4 - L3*d3*m4*theta1_dot*theta3_dot*cos(theta2 + 2*theta3) - L4*d2*m5*theta1_dot*theta2_dot*cos(2*theta2 + theta3) - (L4*d2*m5*theta1_dot*theta3_dot*cos(2*theta2 + theta3))/2 - (L4*d3*m5*theta1_dot*theta2_dot*cos(theta2 + 2*theta3))/2 - (L4*d3*m5*theta2_dot*theta3_dot*cos(theta1 - theta3))/4 - L4*d3*m5*theta1_dot*theta3_dot*cos(theta2 + 2*theta3) + (L2*L3*m4*theta2_dot*theta3_dot*sin(theta1 + theta2 + theta3))/4 + (L2*L4*m5*theta2_dot*theta3_dot*sin(theta1 + theta2 + theta3))/4 - 2*d2*d3*m3*theta1_dot*theta2_dot*sin(theta2 - theta3) + 2*d2*d3*m3*theta1_dot*theta3_dot*sin(theta2 - theta3) - 2*d2*d3*m4*theta1_dot*theta2_dot*sin(theta2 - theta3) + 2*d2*d3*m4*theta1_dot*theta3_dot*sin(theta2 - theta3) - 2*d2*d3*m5*theta1_dot*theta2_dot*sin(theta2 - theta3) + 2*d2*d3*m5*theta1_dot*theta3_dot*sin(theta2 - theta3) + (L2*L3*m4*theta2_dot*theta3_dot*sin(2*theta2 + 2*theta3))/2 - 2*L3*L4*m5*theta1_dot*theta2_dot*sin(2*theta2 + 2*theta3) + (L2*L4*m5*theta2_dot*theta3_dot*sin(2*theta2 + 2*theta3))/2 - 2*L3*L4*m5*theta1_dot*theta3_dot*sin(2*theta2 + 2*theta3) + L3*L4*m5*theta2_dot*theta3_dot*sin(2*theta2 + 2*theta3) + (L2*L3*m4*theta2_dot*theta3_dot*sin(theta2 - theta1 + theta3))/4 + (L2*L4*m5*theta2_dot*theta3_dot*sin(theta2 - theta1 + theta3))/4 - 2*L2*d3*m3*theta1_dot*theta2_dot*cos(theta1 + 2*theta2 + theta3) - L2*d3*m3*theta1_dot*theta3_dot*cos(theta1 + 2*theta2 + theta3) - 2*L2*d4*m4*theta1_dot*theta2_dot*cos(theta1 + 2*theta2 + theta3) - L2*d4*m4*theta1_dot*theta3_dot*cos(theta1 + 2*theta2 + theta3);
                                                                                                                                                                                                                                                                                                                                                                                                                                                                                                                                                                                                                                                                                                                                                                                                                                                                                                                                                                                                                                                                                                                                                                                                                                                                                                                                                                                                                                                                                                                                                                                     (d3^2*m3*theta1_dot^2*sin(theta1 + theta2))/2 - (d2^2*m2*theta1_dot^2*sin(theta1 + theta2))/2 - (L2^2*m3*theta1_dot^2*sin(theta1 + theta2))/4 - (L2^2*m3*theta1_dot^2*sin(theta1 - theta2))/4 - (L2^2*m3*theta2_dot^2*sin(theta1 + theta2 + theta3))/4 - (L2^2*m3*theta3_dot^2*sin(theta1 + theta2 + theta3))/4 - (L3^2*m4*theta1_dot^2*sin(theta1 + theta2 + theta3))/4 - (L3^2*m4*theta2_dot^2*sin(theta1 + theta2 + theta3))/4 - (L3^2*m4*theta3_dot^2*sin(theta1 + theta2 + theta3))/4 - (L4^2*m5*theta1_dot^2*sin(theta1 + theta2 + theta3))/4 - (L4^2*m5*theta2_dot^2*sin(theta1 + theta2 + theta3))/4 - (L4^2*m5*theta3_dot^2*sin(theta1 + theta2 + theta3))/4 - (d2^2*m2*theta1_dot^2*sin(theta1 - theta2))/2 + (L2^2*m3*theta1_dot^2*sin(2*theta2))/2 + (L2^2*m4*theta1_dot^2*sin(2*theta2))/2 + (L2^2*m5*theta1_dot^2*sin(2*theta2))/2 + d4^2*m4*theta1_dot^2*sin(theta1 + theta2 + theta3) + (d2^2*m2*theta1_dot^2*sin(2*theta2))/2 + (L2^2*m3*theta1_dot^2*sin(2*theta2 + 2*theta3))/8 + (5*L3^2*m4*theta1_dot^2*sin(2*theta2 + 2*theta3))/8 + (L3^2*m5*theta1_dot^2*sin(2*theta2 + 2*theta3))/2 + (5*L4^2*m5*theta1_dot^2*sin(2*theta2 + 2*theta3))/8 + (L2^2*m3*theta2_dot^2*sin(theta2 - theta1 + theta3))/4 + (L2^2*m3*theta3_dot^2*sin(theta2 - theta1 + theta3))/4 + (L3^2*m4*theta1_dot^2*sin(theta2 - theta1 + theta3))/4 + (L3^2*m4*theta2_dot^2*sin(theta2 - theta1 + theta3))/4 + (L3^2*m4*theta3_dot^2*sin(theta2 - theta1 + theta3))/4 + (L4^2*m5*theta1_dot^2*sin(theta2 - theta1 + theta3))/4 + (L4^2*m5*theta2_dot^2*sin(theta2 - theta1 + theta3))/4 + (L4^2*m5*theta3_dot^2*sin(theta2 - theta1 + theta3))/4 + (d3^2*m3*theta1_dot^2*sin(theta1 + theta2 + 2*theta3))/2 + (L2^2*m3*theta1_dot*theta3_dot*sin(theta1 + theta2))/4 + (d3*d4*m4*theta1_dot^2*sin(theta1 + theta2))/2 + (L2*d3*m3*theta1_dot^2*cos(theta1))/2 - (L2*d3*m3*theta1_dot^2*cos(theta2))/4 + (L2*d4*m4*theta1_dot^2*cos(theta1))/2 - (L3*d3*m4*theta1_dot^2*cos(theta2))/4 + L3*d4*m4*theta1_dot^2*cos(theta1) - (L4*d3*m5*theta1_dot^2*cos(theta2))/4 + (L4*d4*m5*theta1_dot^2*cos(theta1))/2 - (L2*d3*m3*theta1_dot^2*cos(theta1 + 2*theta2 + 2*theta3))/2 - (L2*d4*m4*theta1_dot^2*cos(theta1 + 2*theta2 + 2*theta3))/2 + (L3*d4*m4*theta1_dot^2*cos(theta1 + 2*theta2 + 2*theta3))/2 + d2*d4*m4*theta1_dot^2*sin(theta2) + d2*d4*m5*theta1_dot^2*sin(theta2) - (L2*L3*m4*theta1_dot^2*sin(theta1 - theta2))/4 - (L2*L4*m5*theta1_dot^2*sin(theta1 - theta2))/4 + L2*L3*m4*theta1_dot^2*sin(2*theta2 + theta3) + L2*L3*m5*theta1_dot^2*sin(2*theta2 + theta3) + L2*L4*m5*theta1_dot^2*sin(2*theta2 + theta3) + (L2*d2*m3*theta1_dot^2*cos(theta1 - theta2))/4 + (L2*d3*m3*theta1_dot^2*cos(theta1 - theta3))/4 + (L3*d2*m4*theta1_dot^2*cos(theta1 - theta2))/4 + (L2*d2*m3*theta1_dot^2*cos(2*theta2 + theta3))/2 + (L2*d3*m3*theta1_dot^2*cos(theta2 + 2*theta3))/4 + (L3*d3*m4*theta1_dot^2*cos(theta1 - theta3))/4 + (L4*d2*m5*theta1_dot^2*cos(theta1 - theta2))/4 + (L3*d2*m4*theta1_dot^2*cos(2*theta2 + theta3))/2 + (L3*d3*m4*theta1_dot^2*cos(theta2 + 2*theta3))/4 + (L4*d3*m5*theta1_dot^2*cos(theta1 - theta3))/4 + (L4*d2*m5*theta1_dot^2*cos(2*theta2 + theta3))/2 + (L4*d3*m5*theta1_dot^2*cos(theta2 + 2*theta3))/4 - (L2*L3*m4*theta2_dot^2*sin(theta1 + theta2 + theta3))/4 - (L2*L3*m4*theta3_dot^2*sin(theta1 + theta2 + theta3))/4 - (L2*L4*m5*theta2_dot^2*sin(theta1 + theta2 + theta3))/4 - (L3*L4*m5*theta1_dot^2*sin(theta1 + theta2 + theta3))/4 - (L2*L4*m5*theta3_dot^2*sin(theta1 + theta2 + theta3))/4 - (L3*L4*m5*theta2_dot^2*sin(theta1 + theta2 + theta3))/4 - (L3*L4*m5*theta3_dot^2*sin(theta1 + theta2 + theta3))/4 - (L2^2*m3*theta1_dot*theta3_dot*sin(theta1 - theta2))/4 + d2*d3*m3*theta1_dot^2*sin(theta2 - theta3) + d2*d3*m4*theta1_dot^2*sin(theta2 - theta3) + d2*d3*m5*theta1_dot^2*sin(theta2 - theta3) - (L2^2*m3*theta1_dot*theta2_dot*sin(theta1 + theta2 + theta3))/2 - (L2^2*m3*theta1_dot*theta3_dot*sin(theta1 + theta2 + theta3))/4 - (L2^2*m3*theta2_dot*theta3_dot*sin(theta1 + theta2 + theta3))/2 - (L3^2*m4*theta1_dot*theta2_dot*sin(theta1 + theta2 + theta3))/2 - (L3^2*m4*theta1_dot*theta3_dot*sin(theta1 + theta2 + theta3))/2 - (L3^2*m4*theta2_dot*theta3_dot*sin(theta1 + theta2 + theta3))/2 - (L4^2*m5*theta1_dot*theta2_dot*sin(theta1 + theta2 + theta3))/2 - (L4^2*m5*theta1_dot*theta3_dot*sin(theta1 + theta2 + theta3))/2 - (L4^2*m5*theta2_dot*theta3_dot*sin(theta1 + theta2 + theta3))/2 + L3*L4*m5*theta1_dot^2*sin(2*theta2 + 2*theta3) + (L2*L3*m4*theta2_dot^2*sin(theta2 - theta1 + theta3))/4 + (L2*L3*m4*theta3_dot^2*sin(theta2 - theta1 + theta3))/4 + (L2*L4*m5*theta2_dot^2*sin(theta2 - theta1 + theta3))/4 + (L3*L4*m5*theta1_dot^2*sin(theta2 - theta1 + theta3))/4 + (L2*L4*m5*theta3_dot^2*sin(theta2 - theta1 + theta3))/4 + (L3*L4*m5*theta2_dot^2*sin(theta2 - theta1 + theta3))/4 + (L3*L4*m5*theta3_dot^2*sin(theta2 - theta1 + theta3))/4 + L2*d3*m3*theta1_dot^2*cos(theta1 + 2*theta2 + theta3) + L2*d4*m4*theta1_dot^2*cos(theta1 + 2*theta2 + theta3) + (L2^2*m3*theta1_dot*theta3_dot*sin(2*theta2 + 2*theta3))/2 - (L2^2*m3*theta1_dot*theta2_dot*sin(theta2 - theta1 + theta3))/2 - (L2^2*m3*theta1_dot*theta3_dot*sin(theta2 - theta1 + theta3))/4 + (L2^2*m3*theta2_dot*theta3_dot*sin(theta2 - theta1 + theta3))/2 - (L3^2*m4*theta1_dot*theta2_dot*sin(theta2 - theta1 + theta3))/2 - (L3^2*m4*theta1_dot*theta3_dot*sin(theta2 - theta1 + theta3))/2 + (L3^2*m4*theta2_dot*theta3_dot*sin(theta2 - theta1 + theta3))/2 - (L4^2*m5*theta1_dot*theta2_dot*sin(theta2 - theta1 + theta3))/2 - (L4^2*m5*theta1_dot*theta3_dot*sin(theta2 - theta1 + theta3))/2 + (L4^2*m5*theta2_dot*theta3_dot*sin(theta2 - theta1 + theta3))/2 - (L2*L3*m4*theta1_dot^2*sin(theta1 + theta2))/4 - (L2*L4*m5*theta1_dot^2*sin(theta1 + theta2))/4 + d2*d3*m3*theta1_dot^2*sin(theta1 + 2*theta2 + theta3) + d2*d4*m4*theta1_dot^2*sin(theta1 + 2*theta2 + theta3) + (d3*d4*m4*theta1_dot^2*sin(theta1 + theta2 + 2*theta3))/2 + (L2*d2*m3*theta1_dot^2*cos(theta1 + theta2))/4 + (L2*d3*m3*theta1_dot^2*cos(theta1 + theta3))/4 + (L3*d2*m4*theta1_dot^2*cos(theta1 + theta2))/4 + (L3*d3*m4*theta1_dot^2*cos(theta1 + theta3))/4 + (L4*d2*m5*theta1_dot^2*cos(theta1 + theta2))/4 + (L4*d3*m5*theta1_dot^2*cos(theta1 + theta3))/4 + (L2*L3*m4*theta1_dot*theta3_dot*sin(theta1 + theta2))/4 + (L2*L4*m5*theta1_dot*theta3_dot*sin(theta1 + theta2))/4 - (L2*d2*m3*theta1_dot*theta3_dot*cos(theta1 + theta2))/4 + (L2*d3*m3*theta1_dot*theta3_dot*cos(theta1 + theta3))/4 - (L3*d2*m4*theta1_dot*theta3_dot*cos(theta1 + theta2))/4 + (L3*d3*m4*theta1_dot*theta3_dot*cos(theta1 + theta3))/4 - (L4*d2*m5*theta1_dot*theta3_dot*cos(theta1 + theta2))/4 - L2*d4*m4*theta1_dot*theta3_dot*cos(theta2 + theta3) - L2*d4*m5*theta1_dot*theta3_dot*cos(theta2 + theta3) + (L4*d3*m5*theta1_dot*theta3_dot*cos(theta1 + theta3))/4 - L2*d2*m3*theta1_dot*theta3_dot*cos(theta3) - L2*d2*m4*theta1_dot*theta3_dot*cos(theta3) - L2*d2*m5*theta1_dot*theta3_dot*cos(theta3) - L3*d2*m4*theta1_dot*theta3_dot*cos(theta3) + L3*d3*m4*theta1_dot*theta3_dot*cos(theta2) - L3*d2*m5*theta1_dot*theta3_dot*cos(theta3) + L3*d3*m5*theta1_dot*theta3_dot*cos(theta2) - L4*d2*m5*theta1_dot*theta3_dot*cos(theta3) + L4*d3*m5*theta1_dot*theta3_dot*cos(theta2) - L2*d3*m3*theta1_dot*theta3_dot*cos(theta1 + 2*theta2 + 2*theta3) - L2*d4*m4*theta1_dot*theta3_dot*cos(theta1 + 2*theta2 + 2*theta3) - (L2*L3*m4*theta1_dot*theta3_dot*sin(theta1 - theta2))/4 - (L2*L4*m5*theta1_dot*theta3_dot*sin(theta1 - theta2))/4 + (L2*d2*m3*theta1_dot*theta3_dot*cos(theta1 - theta2))/4 - (L2*d3*m3*theta1_dot*theta3_dot*cos(theta1 - theta3))/4 + (L3*d2*m4*theta1_dot*theta3_dot*cos(theta1 - theta2))/4 - (L3*d3*m4*theta1_dot*theta3_dot*cos(theta1 - theta3))/4 + (L4*d2*m5*theta1_dot*theta3_dot*cos(theta1 - theta2))/4 - (L4*d3*m5*theta1_dot*theta3_dot*cos(theta1 - theta3))/4 - (L2*L3*m4*theta1_dot*theta2_dot*sin(theta1 + theta2 + theta3))/2 - (L2*L3*m4*theta1_dot*theta3_dot*sin(theta1 + theta2 + theta3))/4 - (L2*L3*m4*theta2_dot*theta3_dot*sin(theta1 + theta2 + theta3))/2 - (L2*L4*m5*theta1_dot*theta2_dot*sin(theta1 + theta2 + theta3))/2 - (L2*L4*m5*theta1_dot*theta3_dot*sin(theta1 + theta2 + theta3))/4 - (L3*L4*m5*theta1_dot*theta2_dot*sin(theta1 + theta2 + theta3))/2 - (L2*L4*m5*theta2_dot*theta3_dot*sin(theta1 + theta2 + theta3))/2 - (L3*L4*m5*theta1_dot*theta3_dot*sin(theta1 + theta2 + theta3))/2 - (L3*L4*m5*theta2_dot*theta3_dot*sin(theta1 + theta2 + theta3))/2 + (L2*L3*m4*theta1_dot*theta3_dot*sin(2*theta2 + 2*theta3))/2 + (L2*L4*m5*theta1_dot*theta3_dot*sin(2*theta2 + 2*theta3))/2 - (L2*L3*m4*theta1_dot*theta2_dot*sin(theta2 - theta1 + theta3))/2 - (L2*L3*m4*theta1_dot*theta3_dot*sin(theta2 - theta1 + theta3))/4 + (L2*L3*m4*theta2_dot*theta3_dot*sin(theta2 - theta1 + theta3))/2 - (L2*L4*m5*theta1_dot*theta2_dot*sin(theta2 - theta1 + theta3))/2 - (L2*L4*m5*theta1_dot*theta3_dot*sin(theta2 - theta1 + theta3))/4 - (L3*L4*m5*theta1_dot*theta2_dot*sin(theta2 - theta1 + theta3))/2 + (L2*L4*m5*theta2_dot*theta3_dot*sin(theta2 - theta1 + theta3))/2 - (L3*L4*m5*theta1_dot*theta3_dot*sin(theta2 - theta1 + theta3))/2 + (L3*L4*m5*theta2_dot*theta3_dot*sin(theta2 - theta1 + theta3))/2;
                                                                                                                                                                                                                                                                                                                                                                                                                                                                                                                                                                                                                                                                                                                                                                                                                                                                                                                                                                                                                                                                                                                                                                                                                                                                                                                                                                                                                                                                                                                                                                                                                                                                                                                                                                                                                                                                                                                                                                                                                                                                                                                                                                                                                                                                                                                                                                                                                                                                                                                                                                                                                                                                                                                                                                                                                                                                                                                                                                                                                                                                                                                                                                                                                                                                                                                                                                                                                         d4^2*m4*theta1_dot^2*sin(theta1 + theta2 + theta3) - (L2^2*m3*theta1_dot^2*sin(theta1 - theta2))/4 - (L3^2*m4*theta1_dot^2*sin(theta1 + theta2 + theta3))/4 - (L3^2*m4*theta2_dot^2*sin(theta1 + theta2 + theta3))/4 - (L3^2*m4*theta3_dot^2*sin(theta1 + theta2 + theta3))/4 - (L4^2*m5*theta1_dot^2*sin(theta1 + theta2 + theta3))/4 - (L4^2*m5*theta2_dot^2*sin(theta1 + theta2 + theta3))/4 - (L4^2*m5*theta3_dot^2*sin(theta1 + theta2 + theta3))/4 - (L2^2*m3*theta1_dot^2*sin(theta1 + theta2))/4 + (L2^2*m3*theta1_dot^2*sin(2*theta2 + 2*theta3))/8 + (5*L3^2*m4*theta1_dot^2*sin(2*theta2 + 2*theta3))/8 + (L3^2*m5*theta1_dot^2*sin(2*theta2 + 2*theta3))/2 + (5*L4^2*m5*theta1_dot^2*sin(2*theta2 + 2*theta3))/8 + (L3^2*m4*theta1_dot^2*sin(theta2 - theta1 + theta3))/4 + (L3^2*m4*theta2_dot^2*sin(theta2 - theta1 + theta3))/4 + (L3^2*m4*theta3_dot^2*sin(theta2 - theta1 + theta3))/4 + (L4^2*m5*theta1_dot^2*sin(theta2 - theta1 + theta3))/4 + (L4^2*m5*theta2_dot^2*sin(theta2 - theta1 + theta3))/4 + (L4^2*m5*theta3_dot^2*sin(theta2 - theta1 + theta3))/4 + d3^2*m3*theta1_dot^2*sin(theta1 + theta2 + 2*theta3) - (L2^2*m3*theta1_dot*theta2_dot*sin(theta1 + theta2))/4 + (L2*L3*m4*theta1_dot^2*sin(theta3))/2 + (L2*L3*m5*theta1_dot^2*sin(theta3))/2 + (L2*L4*m5*theta1_dot^2*sin(theta3))/2 + (d2*d3*m3*theta1_dot^2*sin(theta1 + theta3))/2 + (d2*d4*m4*theta1_dot^2*sin(theta1 + theta3))/2 - (L2*d2*m3*theta1_dot^2*cos(theta3))/4 - (L3*d2*m4*theta1_dot^2*cos(theta3))/4 + L3*d4*m4*theta1_dot^2*cos(theta1) - (L4*d2*m5*theta1_dot^2*cos(theta3))/4 + (L4*d4*m5*theta1_dot^2*cos(theta1))/2 + (L3*d4*m4*theta1_dot^2*cos(theta1 + 2*theta2 + 2*theta3))/2 + d3*d4*m4*theta1_dot^2*sin(theta3) + d3*d4*m5*theta1_dot^2*sin(theta3) - (L2*L3*m4*theta1_dot^2*sin(theta1 - theta2))/4 - (L2*L4*m5*theta1_dot^2*sin(theta1 - theta2))/4 + (L2*L3*m4*theta1_dot^2*sin(2*theta2 + theta3))/2 + (L2*L3*m5*theta1_dot^2*sin(2*theta2 + theta3))/2 + (L2*L4*m5*theta1_dot^2*sin(2*theta2 + theta3))/2 + (L2*d2*m3*theta1_dot^2*cos(theta1 - theta2))/4 + (L2*d3*m3*theta1_dot^2*cos(theta1 - theta3))/4 + (L3*d2*m4*theta1_dot^2*cos(theta1 - theta2))/4 + (L2*d2*m3*theta1_dot^2*cos(2*theta2 + theta3))/4 + (L2*d3*m3*theta1_dot^2*cos(theta2 + 2*theta3))/2 + (L3*d3*m4*theta1_dot^2*cos(theta1 - theta3))/4 + (L4*d2*m5*theta1_dot^2*cos(theta1 - theta2))/4 + (L3*d2*m4*theta1_dot^2*cos(2*theta2 + theta3))/4 + (L3*d3*m4*theta1_dot^2*cos(theta2 + 2*theta3))/2 + (L4*d3*m5*theta1_dot^2*cos(theta1 - theta3))/4 + (L4*d2*m5*theta1_dot^2*cos(2*theta2 + theta3))/4 + (L4*d3*m5*theta1_dot^2*cos(theta2 + 2*theta3))/2 - (L3*L4*m5*theta1_dot^2*sin(theta1 + theta2 + theta3))/4 - (L3*L4*m5*theta2_dot^2*sin(theta1 + theta2 + theta3))/4 - (L3*L4*m5*theta3_dot^2*sin(theta1 + theta2 + theta3))/4 + (L2^2*m3*theta1_dot*theta2_dot*sin(theta1 - theta2))/4 - d2*d3*m3*theta1_dot^2*sin(theta2 - theta3) - d2*d3*m4*theta1_dot^2*sin(theta2 - theta3) - d2*d3*m5*theta1_dot^2*sin(theta2 - theta3) - (L2^2*m3*theta1_dot*theta2_dot*sin(theta1 + theta2 + theta3))/4 - (L3^2*m4*theta1_dot*theta2_dot*sin(theta1 + theta2 + theta3))/2 - (L3^2*m4*theta1_dot*theta3_dot*sin(theta1 + theta2 + theta3))/2 - (L3^2*m4*theta2_dot*theta3_dot*sin(theta1 + theta2 + theta3))/2 - (L4^2*m5*theta1_dot*theta2_dot*sin(theta1 + theta2 + theta3))/2 - (L4^2*m5*theta1_dot*theta3_dot*sin(theta1 + theta2 + theta3))/2 - (L4^2*m5*theta2_dot*theta3_dot*sin(theta1 + theta2 + theta3))/2 + L3*L4*m5*theta1_dot^2*sin(2*theta2 + 2*theta3) + (L3*L4*m5*theta1_dot^2*sin(theta2 - theta1 + theta3))/4 + (L3*L4*m5*theta2_dot^2*sin(theta2 - theta1 + theta3))/4 + (L3*L4*m5*theta3_dot^2*sin(theta2 - theta1 + theta3))/4 + (L2*d3*m3*theta1_dot^2*cos(theta1 + 2*theta2 + theta3))/2 + (L2*d4*m4*theta1_dot^2*cos(theta1 + 2*theta2 + theta3))/2 - (L2^2*m3*theta1_dot*theta2_dot*sin(2*theta2 + 2*theta3))/2 - (L2^2*m3*theta1_dot*theta2_dot*sin(theta2 - theta1 + theta3))/4 - (L3^2*m4*theta1_dot*theta2_dot*sin(theta2 - theta1 + theta3))/2 - (L3^2*m4*theta1_dot*theta3_dot*sin(theta2 - theta1 + theta3))/2 + (L3^2*m4*theta2_dot*theta3_dot*sin(theta2 - theta1 + theta3))/2 - (L4^2*m5*theta1_dot*theta2_dot*sin(theta2 - theta1 + theta3))/2 - (L4^2*m5*theta1_dot*theta3_dot*sin(theta2 - theta1 + theta3))/2 + (L4^2*m5*theta2_dot*theta3_dot*sin(theta2 - theta1 + theta3))/2 - (L2*L3*m4*theta1_dot^2*sin(theta1 + theta2))/4 - (L2*L4*m5*theta1_dot^2*sin(theta1 + theta2))/4 + (d2*d3*m3*theta1_dot^2*sin(theta1 + 2*theta2 + theta3))/2 + (d2*d4*m4*theta1_dot^2*sin(theta1 + 2*theta2 + theta3))/2 + d3*d4*m4*theta1_dot^2*sin(theta1 + theta2 + 2*theta3) + (L2*d2*m3*theta1_dot^2*cos(theta1 + theta2))/4 + (3*L2*d3*m3*theta1_dot^2*cos(theta1 + theta3))/4 + (L3*d2*m4*theta1_dot^2*cos(theta1 + theta2))/4 + (L2*d4*m4*theta1_dot^2*cos(theta1 + theta3))/2 + (L3*d3*m4*theta1_dot^2*cos(theta1 + theta3))/4 + (L4*d2*m5*theta1_dot^2*cos(theta1 + theta2))/4 + (L4*d3*m5*theta1_dot^2*cos(theta1 + theta3))/4 - (L2*L3*m4*theta1_dot*theta2_dot*sin(theta1 + theta2))/4 - (L2*L4*m5*theta1_dot*theta2_dot*sin(theta1 + theta2))/4 + (L2*d2*m3*theta1_dot*theta2_dot*cos(theta1 + theta2))/4 - (L2*d3*m3*theta1_dot*theta2_dot*cos(theta1 + theta3))/4 + (L3*d2*m4*theta1_dot*theta2_dot*cos(theta1 + theta2))/4 - (L3*d3*m4*theta1_dot*theta2_dot*cos(theta1 + theta3))/4 + (L4*d2*m5*theta1_dot*theta2_dot*cos(theta1 + theta2))/4 + L2*d4*m4*theta1_dot*theta2_dot*cos(theta2 + theta3) + L2*d4*m5*theta1_dot*theta2_dot*cos(theta2 + theta3) - (L4*d3*m5*theta1_dot*theta2_dot*cos(theta1 + theta3))/4 + L2*d2*m3*theta1_dot*theta2_dot*cos(theta3) + L2*d2*m4*theta1_dot*theta2_dot*cos(theta3) + L2*d2*m5*theta1_dot*theta2_dot*cos(theta3) + L3*d2*m4*theta1_dot*theta2_dot*cos(theta3) - L3*d3*m4*theta1_dot*theta2_dot*cos(theta2) + L3*d2*m5*theta1_dot*theta2_dot*cos(theta3) - L3*d3*m5*theta1_dot*theta2_dot*cos(theta2) + L4*d2*m5*theta1_dot*theta2_dot*cos(theta3) - L4*d3*m5*theta1_dot*theta2_dot*cos(theta2) + L2*d3*m3*theta1_dot*theta2_dot*cos(theta1 + 2*theta2 + 2*theta3) + L2*d4*m4*theta1_dot*theta2_dot*cos(theta1 + 2*theta2 + 2*theta3) + (L2*L3*m4*theta1_dot*theta2_dot*sin(theta1 - theta2))/4 + (L2*L4*m5*theta1_dot*theta2_dot*sin(theta1 - theta2))/4 - (L2*d2*m3*theta1_dot*theta2_dot*cos(theta1 - theta2))/4 + (L2*d3*m3*theta1_dot*theta2_dot*cos(theta1 - theta3))/4 - (L3*d2*m4*theta1_dot*theta2_dot*cos(theta1 - theta2))/4 + (L3*d3*m4*theta1_dot*theta2_dot*cos(theta1 - theta3))/4 - (L4*d2*m5*theta1_dot*theta2_dot*cos(theta1 - theta2))/4 + (L4*d3*m5*theta1_dot*theta2_dot*cos(theta1 - theta3))/4 - (L2*L3*m4*theta1_dot*theta2_dot*sin(theta1 + theta2 + theta3))/4 - (L2*L4*m5*theta1_dot*theta2_dot*sin(theta1 + theta2 + theta3))/4 - (L3*L4*m5*theta1_dot*theta2_dot*sin(theta1 + theta2 + theta3))/2 - (L3*L4*m5*theta1_dot*theta3_dot*sin(theta1 + theta2 + theta3))/2 - (L3*L4*m5*theta2_dot*theta3_dot*sin(theta1 + theta2 + theta3))/2 - (L2*L3*m4*theta1_dot*theta2_dot*sin(2*theta2 + 2*theta3))/2 - (L2*L4*m5*theta1_dot*theta2_dot*sin(2*theta2 + 2*theta3))/2 - (L2*L3*m4*theta1_dot*theta2_dot*sin(theta2 - theta1 + theta3))/4 - (L2*L4*m5*theta1_dot*theta2_dot*sin(theta2 - theta1 + theta3))/4 - (L3*L4*m5*theta1_dot*theta2_dot*sin(theta2 - theta1 + theta3))/2 - (L3*L4*m5*theta1_dot*theta3_dot*sin(theta2 - theta1 + theta3))/2 + (L3*L4*m5*theta2_dot*theta3_dot*sin(theta2 - theta1 + theta3))/2];
 
end
